simulink library "pmm"  (R2021b)
settings: Solver=VariableStepAuto  StartTime=0.0  StopTime=10.0  RelTol=1e-3
undefined symbols (not defined in the file or in its folder): ENUM_ACMAINRLYSTS_OPEN, ENUM_ACPRECHRGRLYSTS_OPEN, ENUM_B2VRLYSTA_OPEN, ENUM_BMSHVSTS_HVOPEN, ENUM_BRAKEPEDAL_RELEASED, ENUM_CACRLYDEM_CLOSE, ENUM_CACRLYSTS_OPEN, ENUM_CHRGFAULT_ACRLYFAIL, ENUM_CHRGFAULT_BCUHVFAIL, ENUM_CHRGFAULT_BCUNEGFAIL, ENUM_CHRGFAULT_BCUTIMEOUT, ENUM_CHRGFAULT_DCDCENABLE, ENUM_CHRGFAULT_DCDCRLYFAIL, ENUM_CHRGFAULT_HVILFAIL, ENUM_CHRGFAULT_PDUHVFAIL, ENUM_CHRGFAULT_RLYCHKFAIL, ENUM_DCDCEACPCURLYSTA_CLOSED, ENUM_DCDCEACPCURLYSTA_FAILTOCLOSE, ENUM_DCDCEACPCURLYSTA_OPEN, ENUM_DCDCEACPCURLYSTA_WELDED, ENUM_DCDCENABLESTS_READY, ENUM_DCDCRLYSTS_OPEN, ENUM_EHPSRLYDEM_CLOSE, ENUM_EHPSRLYSTS_OPEN, ENUM_FOGRLYENCMD_DISABLE, ENUM_GEARACTUALPOSN_D, ENUM_HVPWROFFREQ_POWEROFF, ENUM_KEYSTATUS_OFF, ENUM_KEYSTATUS_ON, ENUM_KEYSTATUS_START, ENUM_LOWBATTVOLTAGE_NORMAL, ENUM_LOWBATTVOLTAGE_POWERDOWN, ENUM_LOWBATTVOLTAGE_POWERUP, ENUM_MCUHVLOOP_POWEROFF, ENUM_MCUHVLOOPSTS_OPEN, ENUM_MCUMAINRLYSTS_OPEN, ENUM_MCUPRECHRGRLYSTS_OPEN, ENUM_PDFAULT_ACRLYOPEN, ENUM_PDFAULT_BCUDISABLE, ENUM_PDFAULT_DCDCDISABLE, ENUM_PDFAULT_DCDCRLYOPEN, ENUM_PDFAULT_EACDISABLE, ENUM_PDFAULT_EACRLYOPEN, ENUM_PDFAULT_EHPSDISABLE, ENUM_PDFAULT_EHPSRLYOPEN, ENUM_PDFAULT_MCUDISABLE, ENUM_PDFAULT_MCUDISCHRG, ENUM_PDFAULT_MCURLYOPEN, ENUM_PEUSELFCHKSTS_NOFAULT, ENUM_PLUGINSTS_NOPLUGIN, ENUM_PLUGINSTS_PLUGIN, ENUM_PMMMODE_DRIVE, ENUM_PMMMODE_LVBATCHRG, ENUM_PUSTATE_DCDCENABLE, ENUM_PUSTATE_EACPRESCHECK, ENUM_PUSTATE_EHPSENABLE, ENUM_PUSTATE_MCUENABLE, ENUM_PUSTATE_PDUMCURLYCLOSED, ENUM_PUSTATE_POWERUPFAIL, ENUM_TARGETGEAR_REVERSE ... (+126)
libraries: hcu_lib x45, simulink x5, ddm x1, dsc x1
(part 6 of 7)

== stateflow chart pmm/PMM/PowerModeManagement/PMM  ==
  state Sleep
    en:
    VPMM_SysPowerMode_enum = ENUM_PMMMODE_SLEEP;
  state Initialize
    en:
    VPMM_SysPowerMode_enum = ENUM_PMMMODE_INITIALIZE;
    VPMM_IGNRlyClose_flg = FALSE;
    VPMM_IRCRlyClose_flg = FALSE;
    VPMM_PowerUpInhibit_flg = FALSE;
    VPMM_SysInitialTO_flg = FALSE;
    du:
    VPMM_ChrgwakeDebon_cnt += 1;
  state Standby
    en:
    VPMM_SysPowerMode_enum = ENUM_PMMMODE_STANDBY;
    VPMM_PowerUpState_enum = ENUM_PUSTATE_INITIALIZE;
    VPMM_PowerUpFault_enum = ENUM_PUFAULT_NOFAULT;
    VPMM_PowerDownState_enum = ENUM_PDSTATE_MCUDISABLE;
    VPMM_PowerDownFault_enum = ENUM_PDFAULT_NOFAULT;
    VPMM_ChrgState_enum = ENUM_CHRGSTATE_CHECKHVRLYOPEN;
    VPMM_ChrgFault_enum = ENUM_CHRGFAULT_NOFAULT;
    VPMM_PowerUpComplete_flg = FALSE;
    VPMM_PowerDownCompleted_flg = FALSE;
    VPMM_HVSelfChkCompleted_flg = FALSE;
    VPMM_HVSelfChkFail_flg = FALSE;
    VPMM_SysInitialTO_flg = FALSE;
    VPMM_ChrgIntoPwrdown_flg = FALSE;
    VPMM_BattHVDem_enum  = ENUM_BATTHVDEM_POWEROFF;
    VPMM_DCDCRlyDem_enum = ENUM_DCDCRLYDEM_OPEN;
    VPMM_CACRlyDem_enum = ENUM_CACRLYDEM_OPEN;
    VPMM_EHPSRlyDem_enum = ENUM_EHPSRLYDEM_OPEN;
    VPMM_MCUHVLoopDem_enum = ENUM_MCUHVLOOP_POWEROFF;
    VPMM_ACHVLoopDem_enum = ENUM_ACHVLOOP_POWEROFF;
    VPMM_PMMDCDCEnableDem_flg = FALSE;
    VPMM_PMMEACEnableDem_flg = FALSE;
    VPMM_PMMEHPSEnableDem_flg = FALSE;
    VPMM_VCUMCUEn_flg = FALSE;
    VPMM_PowerUpInhibit_flg = FALSE;
    VPMM_DrivelineRelease_enum = ENUM_DRIVELINERELEASE_NOTRELEASE;
    VPMM_ExtTorquePrevent_enum = ENUM_TORQUEPRVENT_NOREQUEST;
    VPMM_HVSysReady_enum = ENUM_HVSYSREADY_NOTREADY;
    VPMM_VCUMCUCtrlMd_enum  = ENUM_MCUCTRLMODE_NONE;
    VPMM_AfterrunCompleted_flg = FALSE;
    (default) -> (junction 1799) : {
        | VPMM_TimeHVSelfChk_s = 0;
        | }
    Standby -> (junction 1799) [order 1]
    (junction 1799) -> (junction 585)
    (junction 585) -> (junction 584) [order 1] : [VINP_ChargeWakeup_flg]
    (junction 584) -> (junction 588) : {
        | VPMM_IRCRlyClose_flg = TRUE;
        | }
    (junction 585) -> (junction 586) [order 2] : {
        | VPMM_IGNRlyClose_flg = TRUE;
        | VPMM_IRCRlyClose_flg = TRUE;
        | }
    (junction 586) -> (junction 587) [order 1] : [VPMM_HVUnitSelfChkCompleted4PU_flg]
    (junction 588) -> (junction 589) [order 1] : [VPMM_HVUnitSelfChkCompleted4Chrg_flg]
    (junction 586) -> (junction 590) [order 2]
    (junction 587) -> (junction 591) : {
        | VPMM_HVSelfChkCompleted4PU_flg =TRUE;
        | }
    (junction 588) -> (junction 1309) [order 2] : {
        | VPMM_TimeHVSelfChk_s += task_time_s;
        | }
    (junction 589) -> (junction 592) : {
        | VPMM_HVSelfChkCompleted4Chrg_flg =TRUE;
        | }
    (junction 591) -> (junction 590)
    (junction 590) -> (junction 596) : {VPMM_TimeHVSelfChk_s += task_time_s;}
    (junction 592) -> (junction 1309)
    (junction 1309) -> (junction 594)
    (junction 594) -> (junction 595) [order 1] : [VPMM_TimeHVSelfChk_s > KPMM_TimeHVSelfChk4Chrg_s]
    (junction 596) -> (junction 597) [order 1] : [VPMM_TimeHVSelfChk_s > KPMM_SysInitialTO_s]
    (junction 594) -> (junction 599) [order 2]
    (junction 595) -> (junction 600) : {
        | VPMM_HVSelfChkFail_flg = TRUE;
        | }
    (junction 596) -> (junction 598) [order 2]
    (junction 597) -> (junction 602) : {
        | VPMM_SysInitialTO_flg = TRUE;
        | }
    (junction 600) -> (junction 599)
    (junction 599) -> (junction 602)
    (junction 602) -> (junction 598)
  state Idle
    en:
    %VPMM_SysPowerMode_enum = ENUM_PMMMODE_IDLE;
    VPMM_PwrOffCompleted_flg = FALSE;
    VPMM_IRCRlyClose_flg =FALSE;
    VPMM_IGNRlyClose_flg = FALSE;
    (default) -> (junction 603) : {
        | VPMM_TimeSysPowerOff_s = 0;
        | }
    Idle -> (junction 603) [order 1]
    (junction 603) -> (junction 604) [order 1] : [((VPMM_TimeSysPowerOff_s > KPMM_Time4Sleep_s) && !VINP_ChargeWakeup_flg) ||...
        |  KPMM_ForceEntrySleep_flg]
    (junction 603) -> (junction 605) [order 2] : {
        | VPMM_TimeSysPowerOff_s += task_time_s;
        | }
    (junction 604) -> (junction 606) : {
        | VPMM_PwrOffCompleted_flg = TRUE;
        | }
    (junction 606) -> (junction 605)
  state Drive
    (default) -> (junction 1819)
    (junction 1819) -> (junction 1821) [order 1] : [VPMM_LVChrgInit2PowerUp_flg || VPMM_LVChrgDCDCDis_flg]
    Drive -> (junction 1819) [order 1]
    (junction 1821) -> (junction 1822) : {
        | VPMM_SysPowerMode_enum = ENUM_PMMMODE_LVBATCHRG;
        | }
    (junction 1819) -> (junction 1823) [order 2] : {
        | VPMM_SysPowerMode_enum = ENUM_PMMMODE_DRIVE;
        | }
    (junction 1822) -> (junction 1823)
    (junction 1823) -> (junction 607)
    (junction 607) -> (junction 608) [order 1] : [(VINP_DCChrgConnectSts_enum ~= ENUM_PLUGINSTS_NOPLUGIN) || (!VINP_MCUIGBTEnFbk_flg) || VPMM_LVChrgInit2PowerUp_flg || VPMM_LVChrgDCDCDis_flg]
    (junction 607) -> (junction 609) [order 2]
    (junction 608) -> (junction 613) : {
        | VPMM_DrivelineRelease_enum = ENUM_DRIVELINERELEASE_NOTRELEASE;
        | }
    (junction 609) -> (junction 610) [order 1] : [VINP_DCChrgConnectSts_enum == ENUM_PLUGINSTS_NOPLUGIN]
    (junction 609) -> (junction 611) [order 2]
    (junction 610) -> (junction 612) : {
        | VPMM_DrivelineRelease_enum = ENUM_DRIVELINERELEASE_RELEASE;
        | }
    (junction 612) -> (junction 611)
    (junction 613) -> (junction 612)
  state Powerdown
    en:
    VPMM_SysPowerMode_enum = ENUM_PMMMODE_POWERDOWN;
    VPMM_HVSysReady_enum = ENUM_HVSYSREADY_NOTREADY;
    VPMM_DrivelineRelease_enum = ENUM_DRIVELINERELEASE_NOTRELEASE;
    VPMM_PowerDownCompleted_flg = FALSE;
    state Initialize
      en:
      VPMM_PowerDownFault_enum = ENUM_PDFAULT_NOFAULT;
      VPMM_PowerDownCompleted_flg = FALSE;
      VPMM_HVSysReady_enum = ENUM_HVSYSREADY_NOTREADY;
      VPMM_DrivelineRelease_enum = ENUM_DRIVELINERELEASE_NOTRELEASE;
      VPMM_MCUDisableCompleted_flg = FALSE;
      VPMM_PDUDisableCompleted_flg = FALSE;
      VPMM_BattPDCompleted_flg = FALSE;
      VPMM_BattPackPDFail_flg = FALSE;
      VPMM_MCUDisChrgCompleted_flg=FALSE;
      VPMM_MCUDisChrgFail_flg = FALSE;
      VPMM_MCUEnDischrgCompleted_flg = FALSE;
      VPMM_MCUEnDischrgFail_flg = FALSE;
      VPMM_MCUPassDischrgFinish_flg = FALSE;
      VPMM_PDURLYOpenFinish_flg = FALSE;
      VPMM_PDURLYOpenFinishFM_flg = FALSE;
      VPMM_ForcedPowerDown4IRC_flg = FALSE;
    state MCUDisable
      en:
      VPMM_PowerDownState_enum = ENUM_PDSTATE_MCUDISABLE;
      VPMM_MCUDisableCompleted_flg = FALSE;
      VPMM_TimeMCUDisable_s = 0;
      (default) -> (junction 773) : {
          | VPMM_VCUMCUEn_flg = FALSE;
          | }
      MCUDisable -> (junction 773) [order 1]
      (junction 773) -> (junction 774) [order 1] : [VINP_MCUIGBTEnFbk_flg == FALSE]
      (junction 773) -> (junction 775) [order 2] : {VPMM_TimeMCUDisable_s += task_time_s}
      (junction 774) -> (junction 779) : {
          | VPMM_MCUDisableCompleted_flg = TRUE;
          | }
      (junction 775) -> (junction 776) [order 1] : [VPMM_TimeMCUDisable_s > KPMM_MCUDisableFailtime_s]
      (junction 776) -> (junction 778) : {
          | VPMM_PowerDownFault_enum = ENUM_PDFAULT_MCUDISABLE;
          | VPMM_MCUDisableCompleted_flg = TRUE;
          | }
      (junction 775) -> (junction 777) [order 2]
      (junction 778) -> (junction 777)
      (junction 779) -> (junction 778)
    state PEUDisable
      en:
      VPMM_PowerDownState_enum = ENUM_PDSTATE_PDUDISABLE;
      VPMM_PDUDisableCompleted_flg = FALSE;
      VPMM_TimePDUDisable_s = 0;
      VPMM_TimePDUDisableWait_s = 0;
      VPMM_DCDCDisableFail_flg = FALSE;
      VPMM_EHPSDisableFail_flg = FALSE;
      VPMM_EACDisableFail_flg = FALSE;
      (default) -> (junction 723) : {
          | VPMM_PMMDCDCEnableDem_flg = FALSE;
          | VPMM_PMMEACEnableDem_flg = FALSE;
          | VPMM_PMMEHPSEnableDem_flg = FALSE;
          | }
      PEUDisable -> (junction 723) [order 1]
      (junction 723) -> (junction 724) [order 1] : [
          |  ((VINP_DCDCEnableStatus_enum == ENUM_DCDCENABLESTS_READY) || (VINP_DCDCEnableStatus_enum == ENUM_DCDCENABLESTS_INITIAL)) &&...
          |  ((VINP_EHPSEnableStatus_enum == ENUM_EHPSENABLESTS_READY)  || (VINP_EHPSEnableStatus_enum == ENUM_EHPSENABLESTS_INITIAL)) &&...
          |  ((VINP_EACEnSta_enum == ENUM_CACENABLESTS_READY) || (VINP_EACEnSta_enum == ENUM_CACENABLESTS_INITIAL))
          | ]
      (junction 723) -> (junction 725) [order 2] : {VPMM_TimePDUDisable_s += task_time_s}
      (junction 724) -> (junction 742) : {
          | VPMM_PDUDisableCompleted_flg = TRUE;
          | }
      (junction 725) -> (junction 726) [order 1] : [VPMM_TimePDUDisable_s > KPMM_PDUDisableFailtime_s]
      (junction 725) -> (junction 739) [order 2]
      (junction 726) -> (junction 727) : {VPMM_TimePDUDisableWait_s += task_time_s}
      (junction 727) -> (junction 1305) [order 1] : [
          |  ((VINP_DCDCEnableStatus_enum == ENUM_DCDCENABLESTS_RUN) ||(VINP_DCDCEnableStatus_enum == ENUM_DCDCENABLESTS_FAULT)) &&...
          |  (VPMM_DCDCDisableFail_flg == FALSE)
          | ]
      (junction 727) -> (junction 729) [order 2]
      (junction 1305) -> (junction 735) : {
          | VPMM_DCDCDisableFail_flg = TRUE;
          | VPMM_PowerDownFault_enum = ENUM_PDFAULT_DCDCDISABLE;
          | }
      (junction 729) -> (junction 1303) [order 1] : [
          | ((VINP_EHPSEnableStatus_enum == ENUM_EHPSENABLESTS_RUN) || (VINP_EHPSEnableStatus_enum == ENUM_EHPSENABLESTS_FAULT)) && ...
          | (VPMM_EHPSDisableFail_flg == FALSE)
          | ]
      (junction 729) -> (junction 731) [order 2]
      (junction 1303) -> (junction 734) : {
          | VPMM_EHPSDisableFail_flg = TRUE;
          | VPMM_PowerDownFault_enum = ENUM_PDFAULT_EHPSDISABLE;
          | }
      (junction 731) -> (junction 732) [order 1] : [
          | ((VINP_EACEnSta_enum == ENUM_CACENABLESTS_RUN) || (VINP_EACEnSta_enum == ENUM_CACENABLESTS_FAULT)) && ...
          | (VPMM_EACDisableFail_flg == FALSE)
          | ]
      (junction 732) -> (junction 733) : {
          | VPMM_EACDisableFail_flg = TRUE;
          | VPMM_PowerDownFault_enum = ENUM_PDFAULT_EACDISABLE;
          | }
      (junction 731) -> (junction 736) [order 2]
      (junction 734) -> (junction 733)
      (junction 735) -> (junction 734)
      (junction 733) -> (junction 736)
      (junction 736) -> (junction 737)
      (junction 737) -> (junction 738) [order 1] : [VPMM_TimePDUDisableWait_s > KPMM_PDUDisableWaitime_s]
      (junction 737) -> (junction 740) [order 2]
      (junction 738) -> (junction 741) : {
          | VPMM_PDUDisableCompleted_flg = TRUE;
          | }
      (junction 740) -> (junction 739)
      (junction 741) -> (junction 740)
      (junction 742) -> (junction 741)
    state HVRelayOpen
      en:
      VPMM_PowerDownState_enum = ENUM_PDSTATE_PDURLYOPEN;
      VPMM_PDURLYOpenFinish_flg = FALSE;
      VPMM_TimeHVRlyOpen_s = 0;
      VPMM_TimeHVRlyOpenWait_s = 0;
      VPMM_PDURLYOpenFail_flg = FALSE;
      VPMM_EHPSRlyOpenFail_flg = FALSE;
      VPMM_ACRlyOpenFail_flg = FALSE;
      VPMM_EACRlyOpenFail_flg = FALSE;
      VPMM_DCDCRlyOpenFail_flg = FALSE;
      VPMM_MainRlyOpenFail_flg = FALSE;
      (default) -> (junction 838) : {
          | VPMM_MCUHVLoopDem_enum = ENUM_MCUHVLOOP_POWEROFF;
          | VPMM_DCDCRlyDem_enum = ENUM_DCDCRLYDEM_OPEN;
          | VPMM_CACRlyDem_enum = ENUM_CACRLYDEM_OPEN;
          | VPMM_EHPSRlyDem_enum = ENUM_EHPSRLYDEM_OPEN;
          | VPMM_ACHVLoopDem_enum = ENUM_ACHVLOOP_POWEROFF;
          | }
      (junction 838) -> (junction 839) [order 1] : [
          | (VINP_MCUHVLoopSts_enum == ENUM_MCUHVLOOPSTS_OPEN &&...
          | VPMM_PDUDCDCRlySta_enum == ENUM_DCDCRLYSTS_OPEN &&...
          | VPMM_PDUEACRlySta_enum == ENUM_CACRLYSTS_OPEN &&...
          | VPMM_PDUEHPSRlySta_enum == ENUM_EHPSRLYSTS_OPEN &&...
          | VINP_PDUACRlySta_enum== ENUM_PDUACRLYSTA_OPEN &&...
          | VINP_PDUACRlySta_enum == ENUM_ACMAINRLYSTS_OPEN &&...
          | VINP_PDUMCUPosRlySta_enum == ENUM_MCUMAINRLYSTS_OPEN) && ...
          | ~VPMM_PDURLYOpenFail_flg
          | ]
      HVRelayOpen -> (junction 838) [order 1]
      (junction 838) -> (junction 840) [order 2] : {
          | VPMM_TimeHVRlyOpen_s += task_time_s;
          | }
      (junction 839) -> (junction 852)
      (junction 840) -> (junction 841) [order 1] : [VPMM_TimeHVRlyOpen_s > KPMM_HVRlyOpenFailtime_s]
      (junction 840) -> (junction 866) [order 2]
      (junction 841) -> (junction 842) : {
          | VPMM_TimeHVRlyOpenWait_s += task_time_s;
          | VPMM_PDURLYOpenFail_flg = TRUE;
          | }
      (junction 842) -> (junction 843) [order 1] : [(VPMM_PDUEHPSRlySta_enum ~= ENUM_EHPSRLYSTS_OPEN) && ...
          |  (VPMM_EHPSRlyOpenFail_flg == FALSE)]
      (junction 842) -> (junction 844) [order 2]
      (junction 843) -> (junction 859) : {
          | VPMM_EHPSRlyOpenFail_flg = TRUE;
          | VPMM_PowerDownFault_enum = ENUM_PDFAULT_EHPSRLYOPEN;
          | }
      (junction 844) -> (junction 845) [order 1] : [((VINP_PDUACRlySta_enum~= ENUM_PDUACRLYSTA_OPEN) || ...
          |   (VINP_PDUACRlySta_enum ~= ENUM_ACMAINRLYSTS_OPEN)) && ...
          |   (VPMM_ACRlyOpenFail_flg == FALSE)]
      (junction 844) -> (junction 846) [order 2]
      (junction 845) -> (junction 858) : {
          | VPMM_ACRlyOpenFail_flg = TRUE;
          | VPMM_PowerDownFault_enum = ENUM_PDFAULT_ACRLYOPEN;
          | }
      (junction 846) -> (junction 847) [order 1] : [(VPMM_PDUEACRlySta_enum ~= ENUM_CACRLYSTS_OPEN) &&...
          |  (VPMM_EACRlyOpenFail_flg == FALSE)]
      (junction 846) -> (junction 848) [order 2]
      (junction 847) -> (junction 857) : {
          | VPMM_EACRlyOpenFail_flg = TRUE;
          | VPMM_PowerDownFault_enum = ENUM_PDFAULT_EACRLYOPEN;
          | }
      (junction 848) -> (junction 849) [order 1] : [(VPMM_PDUDCDCRlySta_enum ~= ENUM_DCDCRLYSTS_OPEN) && ...
          |  (VPMM_DCDCRlyOpenFail_flg == FALSE)]
      (junction 848) -> (junction 850) [order 2]
      (junction 849) -> (junction 856) : {
          | VPMM_DCDCRlyOpenFail_flg = TRUE;
          | VPMM_PowerDownFault_enum = ENUM_PDFAULT_DCDCRLYOPEN;
          | }
      (junction 850) -> (junction 851) [order 1] : [((VINP_MCUHVLoopSts_enum ~= ENUM_MCUHVLOOPSTS_OPEN) || ...
          |  (VINP_PDUMCUPosRlySta_enum ~= ENUM_MCUMAINRLYSTS_OPEN)) && ...
          |  (VPMM_MainRlyOpenFail_flg == FALSE)]
      (junction 850) -> (junction 854) [order 2]
      (junction 851) -> (junction 855) : {
          | VPMM_MainRlyOpenFail_flg = TRUE;
          | VPMM_PowerDownFault_enum = ENUM_PDFAULT_MCURLYOPEN;
          | }
      (junction 852) -> (junction 853) [order 1] : [VPMM_BattPackPDFail_flg]
      (junction 852) -> (junction 868) [order 2] : {
          | VPMM_PDURLYOpenFinish_flg = TRUE;
          | }
      (junction 853) -> (junction 869) : {
          | VPMM_PDURLYOpenFinishFM_flg = TRUE;
          | }
      (junction 855) -> (junction 854)
      (junction 856) -> (junction 855)
      (junction 857) -> (junction 856)
      (junction 858) -> (junction 857)
      (junction 859) -> (junction 858)
      (junction 854) -> (junction 860)
      (junction 860) -> (junction 861) [order 1] : [VPMM_TimeHVRlyOpenWait_s > KPMM_HVRlyOpenFailWT_s]
      (junction 860) -> (junction 867) [order 2]
      (junction 861) -> (junction 862)
      (junction 862) -> (junction 863) [order 1] : [VPMM_BattPackPDFail_flg]
      (junction 862) -> (junction 864) [order 2] : {
          | VPMM_PDURLYOpenFinish_flg = TRUE;
          | }
      (junction 863) -> (junction 865) : {
          | VPMM_PDURLYOpenFinishFM_flg = TRUE;
          | }
      (junction 865) -> (junction 864)
      (junction 868) -> (junction 865)
      (junction 864) -> (junction 867)
      (junction 867) -> (junction 866)
      (junction 869) -> (junction 868)
    state BCUPowerDown
      en:
      VPMM_PowerDownState_enum = ENUM_PDSTATE_BCUPWRDOWN;
      VPMM_BattPDCompleted_flg = FALSE;
      VPMM_BattPackPDFail_flg = FALSE;
      VPMM_TimeBattPD_s = 0;
      (default) -> (junction 750) : {
          | VPMM_BattHVDem_enum  = ENUM_BATTHVDEM_POWEROFF;
          | }
      BCUPowerDown -> (junction 750) [order 1]
      (junction 750) -> (junction 751) [order 1] : [VINP_BMSHVSts_enum == ENUM_BMSHVSTS_HVOPEN]
      (junction 750) -> (junction 752) [order 2] : {
          | VPMM_TimeBattPD_s += task_time_s;
          | }
      (junction 751) -> (junction 756) : {
          | VPMM_BattPDCompleted_flg = TRUE;
          | }
      (junction 752) -> (junction 753) [order 1] : [(VPMM_TimeBattPD_s > KPMM_BattDownFailtime_s)]
      (junction 753) -> (junction 755) : {
          | VPMM_PowerDownFault_enum = ENUM_PDFAULT_BCUDISABLE;
          | VPMM_BattPackPDFail_flg = TRUE;
          | }
      (junction 752) -> (junction 754) [order 2]
      (junction 755) -> (junction 754)
      (junction 756) -> (junction 755)
    state MCUDischarge
      en:
      VPMM_PowerDownState_enum = ENUM_PDSTATE_MCUDISCHRG;
      VPMM_MCUDisChrgCompleted_flg=FALSE;
      VPMM_MCUDisChrgFail_flg = FALSE;
      VPMM_TimeMCUDisChrg_s = 0;
      VPMM_AtvDisChgEnFbkLatch_flg = FALSE;
      (default) -> (junction 1839) : {
          | VPMM_VCUMCUCtrlMd_enum = ENUM_MCUCTRLMODE_ACTDISCHRG;
          | }
      (junction 1839) -> (junction 1841)
      MCUDischarge -> (junction 1841) [order 1]
      (junction 1841) -> (junction 1843) [order 1] : [VPMM_AtvDisChgEnFbk_flg]
      (junction 1841) -> (junction 1847) [order 2]
      (junction 1843) -> (junction 1845) : {
          | VPMM_AtvDisChgEnFbkLatch_flg = TRUE;
          | }
      (junction 1845) -> (junction 1847)
      (junction 1847) -> (junction 757)
      (junction 757) -> (junction 758) [order 1] : [((VINP_MCUInVol_V < KPMM_TargetDchrgVolt_V) && VPMM_AtvDisChgEnFbkLatch_flg )|| VPMM_ChrgIntoPwrdown_flg]
      (junction 757) -> (junction 759) [order 2] : {
          | VPMM_TimeMCUDisChrg_s += task_time_s;
          | }
      (junction 758) -> (junction 763) : {
          | VPMM_VCUMCUCtrlMd_enum = ENUM_MCUCTRLMODE_NONE;
          | VPMM_MCUDisChrgCompleted_flg = TRUE;
          | }
      (junction 759) -> (junction 760) [order 1] : [VPMM_TimeMCUDisChrg_s > KPMM_MCUDisChrgFailtime_s]
      (junction 759) -> (junction 761) [order 2]
      (junction 760) -> (junction 762) : {
          | VPMM_PowerDownFault_enum = ENUM_PDFAULT_MCUDISCHRG;
          | VPMM_VCUMCUCtrlMd_enum = ENUM_MCUCTRLMODE_NONE;
          | VPMM_MCUDisChrgFail_flg = TRUE;
          | }
      (junction 762) -> (junction 761)
      (junction 763) -> (junction 762)
    state MCUDischarge_FailMode
      en:
      VPMM_PowerDownState_enum = ENUM_PDSTATE_MCUDISCHRGFS;
      VPMM_TimeMCUEnDisChrg_s  = 0;
      VPMM_TimeMCUDisable_s = 0;
      VPMM_MCUEnDischrgCompleted_flg = FALSE;
      VPMM_MCUEnDischrgFailCom_flg = FALSE;
      VPMM_MCUEnDischrgFinish_flg = FALSE;
      VPMM_MCUEnFailDis_flg = FALSE;
      (default) -> (junction 819) : {
          | VPMM_VCUMCUEn_flg = TRUE;
          | }
      MCUDischarge_FailMode -> (junction 819) [order 3]
      (junction 819) -> (junction 820) [order 1] : [VINP_MCUInVol_V < KPMM_TargetEnDischrgVolt_V]
      MCUDischarge_FailMode -> (junction 820) [order 1] : [VPMM_MCUEnDischrgFinish_flg == TRUE]
      (junction 819) -> (junction 821) [order 2] : {
          | VPMM_TimeMCUEnDisChrg_s += task_time_s;
          | }
      (junction 820) -> (junction 825) : {
          | VPMM_VCUMCUEn_flg = FALSE;
          | VPMM_MCUEnDischrgFinish_flg = TRUE;
          | }
      MCUDischarge_FailMode -> (junction 821) [order 2] : [VPMM_MCUEnFailDis_flg == TRUE]
      (junction 821) -> (junction 822) [order 1] : [VPMM_TimeMCUEnDisChrg_s > KPMM_MCUEnDischrgFailtime_s]
      (junction 821) -> (junction 831) [order 2]
      (junction 822) -> (junction 823) : {
          | VPMM_VCUMCUEn_flg = FALSE;
          | VPMM_MCUEnFailDis_flg = TRUE;
          | }
      (junction 823) -> (junction 824) [order 1] : [VINP_MCUIGBTEnFbk_flg == FALSE]
      (junction 825) -> (junction 826) [order 1] : [VINP_MCUIGBTEnFbk_flg == FALSE]
      (junction 823) -> (junction 829) [order 2] : {
          | VPMM_TimeMCUDisable_s += task_time_s;
          | }
      (junction 824) -> (junction 834) : {
          | VPMM_MCUEnDischrgFail_flg = TRUE;
          | }
      (junction 825) -> (junction 827) [order 2] : {
          | VPMM_TimeMCUDisable_s += task_time_s;
          | }
      (junction 826) -> (junction 837) : {
          | VPMM_MCUEnDischrgCompleted_flg = TRUE;
          | }
      (junction 827) -> (junction 828) [order 1] : [VPMM_TimeMCUDisable_s > KPMM_MCUDisableFailtime_s]
      (junction 827) -> (junction 835) [order 2]
      (junction 828) -> (junction 836) : {
          | VPMM_PowerDownFault_enum = ENUM_PDFAULT_MCUDISABLE;
          | VPMM_MCUEnDischrgCompleted_flg = TRUE;
          | }
      (junction 829) -> (junction 830) [order 1] : [VPMM_TimeMCUDisable_s > KPMM_MCUDisableFailtime_s]
      (junction 829) -> (junction 832) [order 2]
      (junction 830) -> (junction 833) : {
          | VPMM_PowerDownFault_enum = ENUM_PDFAULT_MCUDISABLE;
          | VPMM_MCUEnDischrgFailCom_flg = TRUE;
          | }
      (junction 832) -> (junction 831)
      (junction 833) -> (junction 832)
      (junction 834) -> (junction 833)
      (junction 835) -> (junction 834)
      (junction 836) -> (junction 835)
      (junction 837) -> (junction 836)
    state BCU_FailMode
      en:
      VPMM_PowerDownState_enum = ENUM_PDSTATE_BCUNEGRLUFS;
      VPMM_MainRlyOpenCompleted_flg = FALSE;
      VPMM_MCUDisChrgFail_flg = FALSE;
      VPMM_TimeMCUDisChrg_s = 0;
      (default) -> (junction 796) : {
          | VPMM_VCUMCUCtrlMd_enum = ENUM_MCUCTRLMODE_ACTDISCHRG;
          | }
      BCU_FailMode -> (junction 796) [order 1]
      (junction 796) -> (junction 797) [order 1] : [VINP_MCUInVol_V < KPMM_TargetDchrgVolt_V]
      (junction 797) -> (junction 802) : {
          | VPMM_VCUMCUCtrlMd_enum = ENUM_MCUCTRLMODE_NONE;
          | VPMM_MCUDisChrgCompleted_flg = TRUE;
          | }
      (junction 796) -> (junction 798) [order 2] : {
          | VPMM_TimeMCUDisChrg_s += task_time_s;
          | }
      (junction 798) -> (junction 799) [order 1] : [VPMM_TimeMCUDisChrg_s > KPMM_MCUDisChrgFSFailtime_s]
      (junction 798) -> (junction 800) [order 2]
      (junction 799) -> (junction 801) : {
          | VPMM_PowerDownFault_enum = ENUM_PDFAULT_MCUDISCHRG;
          | VPMM_VCUMCUCtrlMd_enum = ENUM_MCUCTRLMODE_NONE;
          | VPMM_MCUDisChrgFail_flg = TRUE;
          | }
      (junction 801) -> (junction 800)
      (junction 802) -> (junction 801)
    state MCUPassiveDischrg
      en:
      VPMM_PowerDownState_enum = ENUM_PDSTATE_MCUPASSDISCHRG;
      VPMM_TimeMCUPassDisChrg_s = 0;
      VPMM_MCUPassDischrgFinish_flg = FALSE;
      (default) -> (junction 870)
      MCUPassiveDischrg -> (junction 870) [order 1]
      (junction 870) -> (junction 871) [order 1] : [VINP_MCUInVol_V < KPMM_TargetPassDischrgVolt_V]
      (junction 870) -> (junction 872) [order 2] : {VPMM_TimeMCUPassDisChrg_s += task_time_s}
      (junction 871) -> (junction 876) : {
          | VPMM_MCUPassDischrgFinish_flg = TRUE;
          | }
      (junction 872) -> (junction 873) [order 1] : [VPMM_TimeMCUPassDisChrg_s > KPMM_MCUPassDisChrg_s]
      (junction 872) -> (junction 874) [order 2]
      (junction 873) -> (junction 875) : {
          | VPMM_MCUPassDischrgFinish_flg = TRUE;
          | }
      (junction 875) -> (junction 874)
      (junction 876) -> (junction 875)
    state PowerDownCompleted
      en:
      VPMM_PowerDownState_enum = ENUM_PDSTATE_PDCOMPLETED;
      VPMM_PowerDownCompleted_flg = TRUE;
    state PowerdownFailSafeFinished
      en:
      VPMM_PowerDownState_enum = ENUM_PDSTATE_FSCOMPLETED;
      VPMM_PowerDownCompleted_flg = TRUE;
    (default) -> Powerdown.Initialize
    Powerdown.Initialize -> MCUDisable
    MCUDisable -> PEUDisable [order 1] : [VPMM_MCUDisableCompleted_flg]
    PEUDisable -> BCUPowerDown [order 1] : [VPMM_PDUDisableCompleted_flg]
    BCUPowerDown -> HVRelayOpen [order 1] : [VPMM_BattPackPDFail_flg || VDMM_DTCBMSRlyNoFB_flg]
    BCUPowerDown -> MCUDischarge [order 2] : [VPMM_BattPDCompleted_flg]
    MCUDischarge -> HVRelayOpen [order 2] : [VPMM_MCUDisChrgCompleted_flg ||...
        | VPMM_ChrgState_enum != ENUM_CHRGSTATE_CHECKHVRLYOPEN ||...
        | VPMM_ChrgIntoPwrdown_flg]
    MCUDischarge -> MCUDischarge_FailMode [order 1] : [VPMM_MCUDisChrgFail_flg ||...
        | VDMM_DTCMCUCtrlMdNoFB_flg]
    MCUDischarge_FailMode -> HVRelayOpen [order 2] : [VPMM_MCUEnDischrgCompleted_flg]
    MCUDischarge_FailMode -> MCUPassiveDischrg [order 1] : [VPMM_MCUEnDischrgFailCom_flg ||...
        | VPMM_MCUEnDischrgFail_flg]
    HVRelayOpen -> BCU_FailMode [order 1] : [VPMM_PDURLYOpenFinishFM_flg]
    BCU_FailMode -> MCUPassiveDischrg [order 1] : [VPMM_MCUDisChrgFail_flg]
    MCUPassiveDischrg -> PowerdownFailSafeFinished [order 1] : [VPMM_MCUPassDischrgFinish_flg]
    BCU_FailMode -> PowerdownFailSafeFinished [order 2] : [VPMM_MCUDisChrgCompleted_flg]
    HVRelayOpen -> (junction 1486) [order 2]
    HVRelayOpen -> PowerDownCompleted [order 3] : [VPMM_PDURLYOpenFinish_flg]
    (junction 1486) -> PowerdownFailSafeFinished : [VPMM_PDURLYOpenFinish_flg &&...
        | VPMM_MCUEnDischrgCompleted_flg]
  state Powerup
    en:
    VPMM_SysPowerMode_enum = ENUM_PMMMODE_POWERUP;
    VPMM_PowerUpComplete_flg = FALSE;
    VPMM_HVPwrFail_flg  = FALSE;
    state Initialize
      en:
      VPMM_PowerUpState_enum = ENUM_PUSTATE_DRIVESAFE;
      VPMM_PowerUpFault_enum = ENUM_PUFAULT_NOFAULT;
      VPMM_HVRlyCheckCompleted_flg = FALSE;
      VPMM_BattPUCompleted_flg = FALSE;
      VPMM_EHPSEACReady_flg =FALSE;
      VPMM_MCUPrechrgCompleted_flg = FALSE;
      VPMM_HVSysReady_enum = ENUM_HVSYSREADY_NOTREADY;
      VPMM_DrivelineRelease_enum = ENUM_DRIVELINERELEASE_NOTRELEASE;
      VPMM_PowerUpFail_flg = FALSE;
      VPMM_MCUEnableCompleted_flg = FALSE;
      VPMM_PDULoadPUFault_enum = ENUM_PUFAULT_NOFAULT;
    state AlcLockcheck
      en:
      VPMM_PowerUpState_enum = ENUM_PUSTATE_DRIVESAFE;
      (default) -> (junction 1328) : {
          | VPMM_TimeAlcLockCheck_s = 0;
          | }
      AlcLockcheck -> (junction 1328) [order 1]
      (junction 1328) -> (junction 1329)
      (junction 1329) -> (junction 1330) [order 1] : [VPSA_AlcLockPass_flg]
      (junction 1329) -> (junction 1331) [order 2] : {
          | VPMM_TimeAlcLockCheck_s += task_time_s;
          | }
      (junction 1330) -> (junction 1332) : {
          | VPMM_AlcLockCheckCompleted_flg = TRUE;
          | }
      (junction 1332) -> (junction 1331)
    state HVRlycheck
      en:
      VPMM_PowerUpState_enum = ENUM_PUSTATE_HVRLYCHECK;
      (default) -> (junction 768) : {
          | VPMM_TimeHVRlyCheck_s = 0;
          | VPMM_HVRlyCheckCompleted_flg = FALSE;
          | VPMM_BattHVDem_enum = ENUM_BATTHVDEM_POWEROFF;
          | VPMM_DCDCRlyDem_enum = ENUM_DCDCRLYDEM_OPEN;
          | VPMM_EHPSRlyDem_enum = ENUM_EHPSRLYDEM_OPEN;
          | VPMM_CACRlyDem_enum = ENUM_CACRLYDEM_OPEN;
          | VPMM_MCUHVLoopDem_enum = ENUM_MCUHVLOOP_POWEROFF;
          | VPMM_ACHVLoopDem_enum = ENUM_ACHVLOOP_POWEROFF;
          | }
      HVRlycheck -> (junction 768) [order 1]
      (junction 768) -> (junction 769)
      (junction 769) -> (junction 770) [order 1] : [VPMM_RlyOpenCheck_flg]
      (junction 769) -> (junction 771) [order 2] : {
          | VPMM_TimeHVRlyCheck_s += task_time_s;
          | }
      (junction 770) -> (junction 772) : {
          | VPMM_HVRlyCheckCompleted_flg = TRUE;
          | }
      (junction 772) -> (junction 771)
    state HVPwrUpProcess
      en:
      VPMM_BattPUCompleted_flg = FALSE;
      VPMM_DCDCRlyUpCompleted_flg = FALSE;
      VPMM_PDURelayPUReady_flg = FALSE;
      VPMM_MCUPrechrgCompleted_flg = FALSE;
      VPMM_DCDCEnableCompleted_flg = FALSE;
      VPMM_MCUEnableCompleted_flg  = FALSE;
      VPMM_PowerUpComplete_flg = FALSE;
      VPMM_HVPwrFail_flg  = FALSE;
      VPMM_DCDCEnableProc_flg = FALSE;
      VPMM_MCUPrechrgProc_flg = FALSE;
      VPMM_MCUEnableProc_flg = FALSE;
      VPMM_EHPSEnableProc_flg = FALSE;
      VPMM_CACPresReadyProc_flg = FALSE;
      VPMM_PMMEHPSEnableDem_flg = FALSE;
      VPMM_EHPSEnableCompleted_flg = FALSE;
      VPMM_EHPSIniFinish_flg = FALSE;
      VPMM_PMMEACEnableDem_flg = FALSE;
      VPMM_EACEnableCompleted_flg = FALSE;
      VPMM_AirPressReady_flg = FALSE;
      state BattPackPowerup
        en:
        VPMM_PowerUpState_enum = ENUM_PUSTATE_BCUPOSRLYCLOSED;
        VPMM_BattPUCompleted_flg = FALSE;
        (default) -> (junction 685) : {
            | VPMM_TimeBattPU_s = 0;
            | }
        BattPackPowerup -> (junction 685) [order 1]
        (junction 685) -> (junction 686) : {
            | VPMM_BattHVDem_enum = ENUM_BATTHVDEM_POWERON;
            | }
        (junction 686) -> (junction 687) [order 1] : [VINP_BMSHVSts_enum == ENUM_BMSHVSTS_HVCLOSED]
        (junction 686) -> (junction 688) [order 2] : {
            | VPMM_TimeBattPU_s += task_time_s;
            | }
        (junction 687) -> (junction 689) : {
            | VPMM_BattPUCompleted_flg = TRUE;
            | }
        (junction 689) -> (junction 688)
      state DCDCRlyClosed
        en:
        VPMM_PowerUpState_enum = ENUM_PUSTATE_DCDCRLYCLOSED;
        VPMM_DCDCRlyUpCompleted_flg = FALSE;
        (default) -> (junction 878) : {
            | VPMM_TimeDCDCRlyDemDelay_s = 0;
            | VPMM_TimeDCDCRlyPU_s = 0;
            | }
        Powerup.HVPwrUpProcess.DCDCRlyClosed -> (junction 878) [order 1]
        (junction 878) -> (junction 879) [order 1] : [VPMM_TimeDCDCRlyDemDelay_s > KPMM_DCDCRlyDemDelayTime_s]
        (junction 878) -> (junction 882) [order 2] : {
            | VPMM_TimeDCDCRlyDemDelay_s += task_time_s;
            | }
        (junction 879) -> (junction 880) : {
            | VPMM_DCDCRlyDem_enum = ENUM_DCDCRLYDEM_CLOSE;
            | }
        (junction 880) -> (junction 881) [order 1] : [VPMM_PDUDCDCRlySta_enum == ENUM_DCDCRLYSTS_CLOSED]
        (junction 880) -> (junction 883) [order 2] : {
            | VPMM_TimeDCDCRlyPU_s += task_time_s;
            | }
        (junction 881) -> (junction 884) : {
            | VPMM_DCDCRlyUpCompleted_flg = TRUE;
            | }
        (junction 882) -> (junction 883)
        (junction 884) -> (junction 883)
      state PDULoadRlyClosed
        en:
        VPMM_PowerUpState_enum = ENUM_PUSTATE_PDURLYCLOSED;
        VPMM_CACRlyUpCompleted_flg = FALSE;
        VPMM_EHPSRlyUpCompleted_flg = FALSE;
        VPMM_ACMainRlyUpCompleted_flg = FALSE;
        VPMM_PDURelayPUReady_flg = FALSE;
        (default) -> (junction 885) : {
            | VPMM_TimePDULoadRlyPU_s = 0;
            | }
        PDULoadRlyClosed -> (junction 885) [order 1]
        (junction 885) -> (junction 886) : {
            | VPMM_CACRlyDem_enum = ENUM_CACRLYDEM_CLOSE;
            | VPMM_EHPSRlyDem_enum = ENUM_EHPSRLYDEM_CLOSE;
            | VPMM_ACHVLoopDem_enum = ENUM_ACHVLOOP_POWERON;
            | }
        (junction 886) -> (junction 887) [order 1] : [VPMM_PDUEACRlySta_enum == ENUM_CACRLYSTS_CLOSED]
        (junction 886) -> (junction 888) [order 2]
        (junction 887) -> (junction 889) : {
            | VPMM_CACRlyUpCompleted_flg = TRUE;
            | }
        (junction 889) -> (junction 888)
        (junction 888) -> (junction 890)
        (junction 890) -> (junction 891) [order 1] : [VPMM_PDUEHPSRlySta_enum == ENUM_EHPSRLYSTS_CLOSED]
        (junction 890) -> (junction 892) [order 2]
        (junction 891) -> (junction 893) : {
            | VPMM_EHPSRlyUpCompleted_flg = TRUE;
            | }
        (junction 893) -> (junction 892)
        (junction 892) -> (junction 894)
        (junction 894) -> (junction 895) [order 1] : [VINP_PDUACRlySta_enum ==ENUM_PDUACRLYSTA_CLOSE]
        (junction 894) -> (junction 896) [order 2]
        (junction 895) -> (junction 897) : {
            | VPMM_ACMainRlyUpCompleted_flg = TRUE;
            | }
        (junction 897) -> (junction 896)
        (junction 896) -> (junction 898)
        (junction 898) -> (junction 899) [order 1] : [VPMM_ACMainRlyUpCompleted_flg && VPMM_EHPSRlyUpCompleted_flg && VPMM_CACRlyUpCompleted_flg]
        (junction 898) -> (junction 900) [order 2] : {
            | VPMM_TimePDULoadRlyPU_s += task_time_s;
            | }
        (junction 899) -> (junction 901) : {
            | VPMM_PDURelayPUReady_flg = TRUE;
            | }
        (junction 901) -> (junction 900)
        (junction 900) -> (junction 902)
      state HVPwrEnable
        state MCU [parallel]
          settings: executionOrder=1
          state MCUPrechrg
            en:
            VPMM_MCUPrechrgCompleted_flg = FALSE;
            VPMM_PowerUpState_enum = ENUM_PUSTATE_PDUMCURLYCLOSED;
            VPMM_MCUPrechrgProc_flg = TRUE;
            exit:
            VPMM_MCUPrechrgProc_flg = FALSE;
            (default) -> (junction 908) : {
                | VPMM_TimeMCUPrechrgRlyPU_s = 0;
                | }
            MCUPrechrg -> (junction 908) [order 1]
            (junction 908) -> (junction 909) [order 1] : [VINP_MCUFailGrade_enum == ZERO_INT]
            (junction 909) -> (junction 910) : {
                | VPMM_MCUHVLoopDem_enum = ENUM_MCUHVLOOP_POWERON;
                | }
            (junction 908) -> (junction 912) [order 2] : {
                | VPMM_TimeMCUPrechrgRlyPU_s += task_time_s;
                | }
            (junction 910) -> (junction 911) [order 1] : [VINP_MCUHVLoopSts_enum == ENUM_MCUHVLOOPSTS_PRECHARGEFIN]
            (junction 911) -> (junction 914) : {
                | VPMM_MCUPrechrgCompleted_flg = TRUE;
                | }
            (junction 910) -> (junction 913) [order 2] : {
                | VPMM_TimeMCUPrechrgRlyPU_s += task_time_s;
                | }
            (junction 913) -> (junction 912)
            (junction 914) -> (junction 913)
          state MCUEnable
            en:
            VPMM_MCUEnableCompleted_flg  = FALSE;
            VPMM_PowerUpState_enum = ENUM_PUSTATE_MCUENABLE;
            VPMM_MCUEnableProc_flg = TRUE;
            exit:
            VPMM_MCUEnableProc_flg = FALSE;
            (default) -> (junction 704) : {
                | VPMM_TimeMCUEnable_s = 0;
                | }
            MCUEnable -> (junction 704)
            (junction 704) -> (junction 705) : {
                | VPMM_VCUMCUEn_flg = TRUE;
                | }
            (junction 705) -> (junction 706) [order 1] : [VINP_MCUIGBTEnFbk_flg == TRUE]
            (junction 705) -> (junction 707) [order 2] : {
                | VPMM_TimeMCUEnable_s += task_time_s;
                | }
            (junction 706) -> (junction 708) : {
                | VPMM_MCUEnableProc_flg = FALSE;
                | VPMM_MCUEnableCompleted_flg = TRUE;
                | }
            (junction 708) -> (junction 707)
          (default) -> MCUPrechrg
          MCUPrechrg -> MCUEnable [order 1] : [VPMM_MCUPrechrgCompleted_flg]
        state PDU [parallel]
          settings: executionOrder=2
          state DCDC
            en:
            VPMM_DCDCEnableCompleted_flg = FALSE;
            VPMM_PowerUpState_enum = ENUM_PUSTATE_DCDCENABLE;
            VPMM_DCDCEnableProc_flg = TRUE;
            exit:
            VPMM_DCDCEnableProc_flg = FALSE;
            (default) -> (junction 903) : {
                | VPMM_TimeDCDCEnable_s = 0;
                | }
            DCDC -> (junction 903) [order 1]
            (junction 903) -> (junction 904) : {
                | VPMM_PMMDCDCEnableDem_flg = TRUE;
                | }
            (junction 904) -> (junction 905) [order 1] : [VINP_DCDCEnableStatus_enum == ENUM_DCDCENABLESTS_RUN]
            (junction 904) -> (junction 906) [order 2] : {
                | VPMM_TimeDCDCEnable_s += task_time_s;
                | }
            (junction 905) -> (junction 907) : {
                | VPMM_DCDCEnableCompleted_flg = TRUE;
                | }
            (junction 907) -> (junction 906)
          state EHPS
            en:
            VPMM_PowerUpState_enum = ENUM_PUSTATE_EHPSENABLE;
            VPMM_EHPSEnableProc_flg = TRUE;
            VPMM_TimeEHPSEnable_s = 0;
            VPMM_TimeEHPSIni_s = 0;
            VPMM_PMMEHPSDemSpd_rpm = 0;
            exit:
            VPMM_EHPSEnableProc_flg = FALSE;
            VPMM_PMMEHPSEnableDem_flg = FALSE;
            VPMM_PMMEHPSDemSpd_rpm = 0;
            (default) -> (junction 1355) : {
                | VPMM_PMMEHPSEnableDem_flg = TRUE;
                | }
            EHPS -> (junction 1355) [order 2]
            (junction 1355) -> (junction 1356) [order 1] : [VINP_EHPSEnableStatus_enum == ENUM_EHPSENABLESTS_RUN]
            EHPS -> (junction 1356) [order 1] : [VPMM_EHPSEnableCompleted_flg == TRUE]
            (junction 1355) -> (junction 1357) [order 2] : {
                | VPMM_TimeEHPSEnable_s += task_time_s;
                | }
            (junction 1356) -> (junction 1366) : {
                | VPMM_EHPSEnableCompleted_flg = TRUE;
                | VPMM_PMMEHPSDemSpd_rpm = KPMM_EHPSSpdDem_rpm;
                | }
            (junction 1366) -> (junction 1368) [order 1] : [VPMM_EHPSIniReady_flg == TRUE]
            (junction 1366) -> (junction 1358) [order 2] : {
                | VPMM_TimeEHPSIni_s += task_time_s;
                | }
            (junction 1368) -> (junction 1370) : {
                | VPMM_EHPSIniFinish_flg = TRUE;
                | }
            (junction 1358) -> (junction 1357)
            (junction 1370) -> (junction 1358)
          state EAC
            en:
            VPMM_PowerUpState_enum = ENUM_PUSTATE_EACPRESCHECK;
            VPMM_CACPresReadyProc_flg = TRUE;
            VPMM_TimeEACEnable_s = 0;
            VPMM_TimeWaitAirPress_s = 0;
            exit:
            VPMM_PMMEACEnableDem_flg = FALSE;
            VPMM_CACPresReadyProc_flg = FALSE;
            (default) -> (junction 1377) : {
                | VPMM_PMMEACEnableDem_flg = TRUE;
                | }
            EAC -> (junction 1377) [order 2]
            (junction 1377) -> (junction 1378) [order 1] : [VINP_EACEnSta_enum == ENUM_CACENABLESTS_RUN]
            EAC -> (junction 1378) [order 1] : [VPMM_EACEnableCompleted_flg]
            (junction 1377) -> (junction 1381) [order 2] : {
                | VPMM_TimeEACEnable_s += task_time_s;
                | }
            (junction 1378) -> (junction 1420) : {
                | VPMM_EACEnableCompleted_flg = TRUE;
                | VPMM_PMMEACEnableDem_flg = FALSE;
                | }
            (junction 1420) -> (junction 1422) [order 1] : [VACC_CACPresReady_flg]
            (junction 1420) -> (junction 1382) [order 2] : {
                | VPMM_TimeWaitAirPress_s += task_time_s;
                | }
            (junction 1422) -> (junction 1424) : {
                | VPMM_AirPressReady_flg = TRUE;
                | }
            (junction 1382) -> (junction 1381)
            (junction 1424) -> (junction 1382)
          (default) -> DCDC
          DCDC -> EHPS [order 1] : [VPMM_DCDCEnableCompleted_flg]
          EHPS -> EAC [order 1] : [VPMM_EHPSIniFinish_flg]
      state FindFaultRoot2
        en:
        VPMM_PDULoadPUFault_enum = ENUM_PUFAULT_NOFAULT;
        (default) -> (junction 809)
        (junction 809) -> (junction 810) [order 1] : [VPMM_PDUEACRlySta_enum ~= ENUM_CACRLYSTS_CLOSED]
        (junction 809) -> (junction 811) [order 2]
        (junction 810) -> (junction 818) : {
            | VPMM_PDULoadPUFault_enum = ENUM_PUFAULT_CACRLYUPFAIL;
            | }
        (junction 811) -> (junction 812) [order 1] : [VPMM_PDUEHPSRlySta_enum ~= ENUM_EHPSRLYSTS_CLOSED]
        (junction 811) -> (junction 813) [order 2]
        (junction 812) -> (junction 817) : {
            | VPMM_PDULoadPUFault_enum = ENUM_PUFAULT_EHPSRLYUPFAIL;
            | }
        (junction 813) -> (junction 814) [order 1] : [VINP_PDUACRlySta_enum ~= ENUM_PDUACRLYSTA_CLOSE]
        (junction 813) -> (junction 815) [order 2]
        (junction 814) -> (junction 816) : {
            | VPMM_PDULoadPUFault_enum = ENUM_PUFAULT_ACMAINRLYUPFAIL;
            | }
        (junction 816) -> (junction 815)
        (junction 817) -> (junction 816)
        (junction 818) -> (junction 817)
      state FindFaultRoot1
        en:
        (default) -> (junction 764)
        (junction 764) -> (junction 765) [order 1] : [(VPMM_TimeEHPSEnable_s > KPMM_EHPSENTimeout_s) || ...
            |  (VPMM_TimeEHPSIni_s > KPMM_EHPSIniTimeout_s)]
        (junction 764) -> (junction 766) [order 2] : {
            | VPMM_PowerUpFault_enum = ENUM_PUFAULT_AIRPRESS;
            | }
        (junction 765) -> (junction 767) : {
            | VPMM_PowerUpFault_enum = ENUM_PUFAULT_EHPSENABLEFAIL;
            | }
        (junction 767) -> (junction 766)
      state HVPwrReady
        en:
        VPMM_PowerUpState_enum = ENUM_PUSTATE_COMPLETED;
        VPMM_PowerUpComplete_flg = TRUE;
        VPMM_HVSysReady_enum = ENUM_HVSYSREADY_READY;
      state HVPwrFail
        en:
        VPMM_HVPwrFail_flg = TRUE;
      (default) -> BattPackPowerup
      BattPackPowerup -> (junction 743) [order 1] : [(VPMM_TimeBattPU_s > KPMM_BattUpFailtime_s) ||...
          | (VINP_BMSHVSts_enum == ENUM_BMSHVSTS_FAILTOHVON) ]
      (junction 743) -> HVPwrFail : {
          | VPMM_PowerUpFault_enum = ENUM_PUFAULT_BATTUPFAIL;
          | }
      BattPackPowerup -> Powerup.HVPwrUpProcess.DCDCRlyClosed [order 2] : [VPMM_BattPUCompleted_flg]
      Powerup.HVPwrUpProcess.DCDCRlyClosed -> (junction 744) [order 1] : [(VPMM_TimeDCDCRlyPU_s > KPMM_DCDCRlyUpFailtime_s) ||...
          | (VPMM_PDUDCDCRlySta_enum ==ENUM_DCDCRLYSTS_FAILTOCLOSE) ]
      (junction 744) -> HVPwrFail : {
          | VPMM_PowerUpFault_enum = ENUM_PUFAULT_DCDCRLYUPFAIL;
          | }
      Powerup.HVPwrUpProcess.DCDCRlyClosed -> PDULoadRlyClosed [order 2] : [VPMM_DCDCRlyUpCompleted_flg]
      PDULoadRlyClosed -> (junction 745) [order 1] : [(VPMM_TimePDULoadRlyPU_s > KPMM_PDULoadRlyPUFailtime_s) ||...
          |  (VPMM_PDUEACRlySta_enum == ENUM_CACRLYSTS_FAILTOCLOSE) ||...
          |  (VPMM_PDUEHPSRlySta_enum == ENUM_EHPSRLYSTS_FAILTOCLOSE) ||...
          |  (VINP_PDUACRlySta_enum== ENUM_PDUACRLYSTA_CLOSEFAILURE)]
      (junction 745) -> FindFaultRoot2
      PDULoadRlyClosed -> HVPwrEnable [order 2] : [VPMM_PDURelayPUReady_flg]
      HVPwrEnable -> (junction 746) [order 1] : [(VPMM_TimeMCUPrechrgRlyPU_s > KPMM_MCUPrechrgFailtime_s) ||...
          |  (VINP_MCUHVLoopSts_enum == ENUM_MCUHVLOOPSTS_FAILED) || ...
          |  (VINP_MCUFailGrade_enum ~= ZERO_INT)]
      (junction 746) -> HVPwrFail : {
          | VPMM_PowerUpFault_enum = ENUM_PUFAULT_MCUPRECHRGFAIL;
          | }
      HVPwrEnable -> (junction 747) [order 2] : [VPMM_TimeMCUEnable_s > KPMM_MCUEnableFailtime_s]
      (junction 747) -> HVPwrFail : {
          | VPMM_PowerUpFault_enum = ENUM_PUFAULT_MCUENABLEFAIL;
          | }
      HVPwrEnable -> (junction 748) [order 3] : [(VPMM_TimeDCDCEnable_s > KPMM_DCDCEnableFailtime_s) ||...
          | (VINP_DCDCEnableStatus_enum == ENUM_DCDCENABLESTS_FAULT)]
      FindFaultRoot2 -> HVPwrFail : {
          | VPMM_PowerUpFault_enum = VPMM_PDULoadPUFault_enum;
          | }
      (junction 748) -> HVPwrFail : {VPMM_PowerUpFault_enum = ENUM_PUFAULT_DCDCENABLEFAIL}
      HVPwrEnable -> (junction 749) [order 4] : [(VPMM_TimeEHPSEnable_s > KPMM_EHPSENTimeout_s) || ...
          |  (VPMM_TimeEHPSIni_s > KPMM_EHPSIniTimeout_s) || ...
          |  (VPMM_TimeEACEnable_s > KPMM_EACENTimeout_s) || ...
          |  (VPMM_TimeWaitAirPress_s > KPMM_WaitAirPressTimeout_s)]
      (junction 749) -> FindFaultRoot1
      HVPwrEnable -> HVPwrReady [order 5] : [VPMM_AirPressReady_flg && VPMM_MCUEnableCompleted_flg ]
      FindFaultRoot1 -> HVPwrFail
    state Timeout
      en:
      VPMM_PowerUpState_enum = ENUM_PUSTATE_POWERUPFAIL;
      VPMM_BattHVDem_enum = ENUM_BATTHVDEM_POWEROFF;
      VPMM_MCUHVLoopDem_enum = ENUM_MCUHVLOOP_POWEROFF;
      VPMM_PMMDCDCEnableDem_flg = FALSE;
      VPMM_DCDCRlyDem_enum = ENUM_DCDCRLYDEM_OPEN;
      VPMM_EHPSRlyDem_enum = ENUM_EHPSRLYDEM_OPEN;
      VPMM_CACRlyDem_enum = ENUM_CACRLYDEM_OPEN;
      VPMM_ACHVLoopDem_enum = ENUM_ACHVLOOP_POWEROFF;
      VPMM_VCUMCUEn_flg = FALSE;
      VPMM_PowerUpFail_flg = TRUE;
    (default) -> Powerup.Initialize
    Powerup.Initialize -> AlcLockcheck
    AlcLockcheck -> (junction 1343) [order 1] : [(VPMM_TimeAlcLockCheck_s > KPMM_AlcLockCheckFailtime_s)]
    (junction 1343) -> Timeout : {
        | VPMM_PowerUpFault_enum = ENUM_PUFAULT_ALINTERLOCK;
        | }
    AlcLockcheck -> HVRlycheck [order 2] : [VPMM_AlcLockCheckCompleted_flg]
    HVRlycheck -> (junction 877) [order 1] : [(VPMM_TimeHVRlyCheck_s > KPMM_HVRlyCheckFailtime_s)]
    (junction 877) -> Timeout : {
        | VPMM_PowerUpFault_enum = ENUM_PUFAULT_HVRLYCHKFAIL;
        | }
    HVRlycheck -> HVPwrUpProcess [order 2] : [VPMM_HVRlyCheckCompleted_flg]
    HVPwrUpProcess -> Timeout : [VPMM_HVPwrFail_flg]
  state Charge
    en:
    VPMM_SysPowerMode_enum = ENUM_PMMMODE_CHARGE;
    VPMM_ChrgIntoPwrdown_flg = FALSE;
    VPMM_PowerUpInhibit_flg = TRUE;
    VPMM_ChrgPowerUpFail_flg = FALSE;
    VPMM_HVRlyCheckCompleted_flg = FALSE;
    VPMM_ChrgPowerUpFail_flg = FALSE;
    VPMM_BattPUCompleted_flg = FALSE;
    VPMM_DCDCRlyUpCompleted_flg = FALSE;
    VPMM_ACMainRlyUpCompleted_flg = FALSE;
    VPMM_DCDCEnableCompleted_flg = FALSE;
    VPMM_CheckChrgStaFail_flg = FALSE;
    VPMM_CheckChrgSta_flg = FALSE;
    VPMM_DCDCNotEnaInChrg_flg =FALSE;
    VPMM_ChrgFinishComplete_flg = FALSE;
    VPMM_BattHVDem_enum = ENUM_BATTHVDEM_POWEROFF;
    VPMM_DCDCRlyDem_enum = ENUM_DCDCRLYDEM_OPEN;
    VPMM_EHPSRlyDem_enum = ENUM_EHPSRLYDEM_OPEN;
    VPMM_CACRlyDem_enum = ENUM_CACRLYDEM_OPEN;
    VPMM_MCUHVLoopDem_enum = ENUM_MCUHVLOOP_POWEROFF;
    VPMM_ACHVLoopDem_enum = ENUM_ACHVLOOP_POWEROFF;
    state HVRlyCheck
      en:
      VPMM_ChrgState_enum = ENUM_CHRGSTATE_CHECKHVRLYOPEN;
      VPMM_HVRlyCheckCompleted_flg = FALSE;
      VPMM_ChrgPowerUpFail_flg = FALSE;
      VPMM_TimeHVRlyCheck_s = 0;
      (default) -> (junction 697) : {
          | VPMM_HVRlyCheckCompleted_flg = FALSE;
          | VPMM_BattHVDem_enum = ENUM_BATTHVDEM_POWEROFF;
          | VPMM_DCDCRlyDem_enum = ENUM_DCDCRLYDEM_OPEN;
          | VPMM_EHPSRlyDem_enum = ENUM_EHPSRLYDEM_OPEN;
          | VPMM_CACRlyDem_enum = ENUM_CACRLYDEM_OPEN;
          | VPMM_MCUHVLoopDem_enum = ENUM_MCUHVLOOP_POWEROFF;
          | VPMM_ACHVLoopDem_enum = ENUM_ACHVLOOP_POWEROFF;
          | }
      HVRlyCheck -> (junction 697) [order 1]
      (junction 697) -> (junction 698) [order 1] : [VPMM_RlyOpenCheck_flg]
      (junction 697) -> (junction 699) [order 2]
      (junction 698) -> (junction 703) : {
          | VPMM_HVRlyCheckCompleted_flg = TRUE;
          | }
      (junction 699) -> (junction 700) [order 1] : [VPMM_TimeHVRlyCheck_s > KPMM_HVRlyCheckFailtime_s]
      (junction 699) -> (junction 701) [order 2] : {
          | VPMM_TimeHVRlyCheck_s += task_time_s;
          | }
      (junction 700) -> (junction 702) : {
          | VPMM_ChrgFault_enum = ENUM_CHRGFAULT_RLYCHKFAIL;
          | VPMM_ChrgPowerUpFail_flg = TRUE;
          | }
      (junction 702) -> (junction 701)
      (junction 703) -> (junction 702)
    state BCUPowerUp
      en:
      VPMM_ChrgState_enum = ENUM_CHRGSTATE_BCUNEGRLYCLOSED;
      VPMM_BattPUCompleted_flg = FALSE;
      VPMM_ChrgPowerUpFail_flg = FALSE;
      VPMM_TimeBattPU_s = 0;
      (default) -> (junction 652) : {
          | VPMM_BattHVDem_enum = ENUM_BATTHVDEM_POWERON;
          | }
      BCUPowerUp -> (junction 652) [order 1]
      (junction 652) -> (junction 653) [order 1] : [VINP_BMSHVSts_enum ==ENUM_BMSHVSTS_HVCLOSED]
      (junction 652) -> (junction 654) [order 2]
      (junction 653) -> (junction 658) : {
          | VPMM_BattPUCompleted_flg = TRUE;
          | }
      (junction 654) -> (junction 655) [order 1] : [(VPMM_TimeBattPU_s > KPMM_BattUpFailtime_s) ||...
          |  (VINP_BMSHVSts_enum == ENUM_BMSHVSTS_FAILTOHVON)]
      (junction 654) -> (junction 656) [order 2] : {
          | VPMM_TimeBattPU_s += task_time_s;
          | }
      (junction 655) -> (junction 657) : {
          | VPMM_ChrgFault_enum = ENUM_CHRGFAULT_BCUNEGFAIL;
          | VPMM_ChrgPowerUpFail_flg = TRUE;
          | }
      (junction 657) -> (junction 656)
      (junction 658) -> (junction 657)
    state DCDCRlyClosed
      en:
      VPMM_ChrgState_enum = ENUM_CHRGSTATE_DCDCRLYCLOSED;
      VPMM_DCDCRlyUpCompleted_flg = FALSE;
      VPMM_ChrgPowerUpFail_flg = FALSE;
      VPMM_TimeDCDCRlyDemDelay_s = 0;
      VPMM_TimeDCDCRlyPU_s = 0;
      (default) -> (junction 614)
      Charge.DCDCRlyClosed -> (junction 614) [order 1]
      (junction 614) -> (junction 615) [order 1] : [VPMM_TimeDCDCRlyDemDelay_s > KPMM_DCDCRlyDemDelayTime_s]
      (junction 614) -> (junction 620) [order 2] : {
          | VPMM_TimeDCDCRlyDemDelay_s += task_time_s;
          | }
      (junction 615) -> (junction 616) : {
          | VPMM_DCDCRlyDem_enum = ENUM_DCDCRLYDEM_CLOSE;
          | }
      (junction 616) -> (junction 617) [order 1] : [VPMM_PDUDCDCRlySta_enum == ENUM_DCDCRLYSTS_CLOSED]
      (junction 616) -> (junction 618) [order 2]
      (junction 617) -> (junction 623) : {
          | VPMM_DCDCRlyUpCompleted_flg = TRUE;
          | }
      (junction 618) -> (junction 619) [order 1] : [(VPMM_TimeDCDCRlyPU_s > KPMM_DCDCRlyUpFailtime_s) ||...
          | (VPMM_PDUDCDCRlySta_enum ==ENUM_DCDCRLYSTS_FAILTOCLOSE) ]
      (junction 618) -> (junction 621) [order 2] : {
          | VPMM_TimeDCDCRlyPU_s += task_time_s;
          | }
      (junction 619) -> (junction 622) : {
          | VPMM_ChrgFault_enum = ENUM_CHRGFAULT_DCDCRLYFAIL;
          | VPMM_ChrgPowerUpFail_flg = TRUE;
          | }
      (junction 620) -> (junction 621)
      (junction 622) -> (junction 621)
      (junction 623) -> (junction 622)
    state ACHVPowerUp
      en:
      VPMM_ChrgState_enum = ENUM_CHRGSTATE_ACRLYCLOSED;
      VPMM_ACMainRlyUpCompleted_flg = FALSE;
      VPMM_ChrgPowerUpFail_flg = FALSE;
      VPMM_TimeACMainRlyPU_s = 0;
      (default) -> (junction 690) : {
          | VPMM_ACHVLoopDem_enum = ENUM_ACHVLOOP_POWERON;
          | }
      ACHVPowerUp -> (junction 690) [order 1]
      (junction 690) -> (junction 691) [order 1] : [VINP_PDUACRlySta_enum== ENUM_PDUACRLYSTA_CLOSE]
      (junction 690) -> (junction 692) [order 2]
      (junction 691) -> (junction 696) : {
          | VPMM_ACMainRlyUpCompleted_flg = TRUE;
          | }
      (junction 692) -> (junction 693) [order 1] : [(VPMM_TimeACMainRlyPU_s > KPMM_ACMainRlyUpFailtime_s) ||...
          |  (VINP_PDUACRlySta_enum== ENUM_PDUACRLYSTA_CLOSEFAILURE) ]
      (junction 692) -> (junction 694) [order 2] : {
          | VPMM_TimeACMainRlyPU_s += task_time_s;
          | }
      (junction 693) -> (junction 695) : {
          | VPMM_ChrgFault_enum = ENUM_CHRGFAULT_ACRLYFAIL;
          | VPMM_ChrgPowerUpFail_flg = TRUE;
          | }
      (junction 695) -> (junction 694)
      (junction 696) -> (junction 695)
    state DCDCEnable
      en:
      VPMM_ChrgState_enum = ENUM_CHRGSTATE_DCDCENABLE;
      VPMM_DCDCEnableCompleted_flg = FALSE;
      VPMM_ChrgPowerUpFail_flg = FALSE;
      VPMM_TimeDCDCEnable_s = 0;
      (default) -> (junction 624) : {
          | VPMM_PMMDCDCEnableDem_flg = TRUE;
          | }
      DCDCEnable -> (junction 624) [order 1]
      (junction 624) -> (junction 625) [order 1] : [VINP_DCDCEnableStatus_enum == ENUM_DCDCENABLESTS_RUN]
      (junction 624) -> (junction 626) [order 2]
      (junction 625) -> (junction 630) : {
          | VPMM_DCDCEnableCompleted_flg = TRUE;
          | }
      (junction 626) -> (junction 627) [order 1] : [(VPMM_TimeDCDCEnable_s > KPMM_DCDCEnableFailtime_s) ||...
          | (VINP_DCDCEnableStatus_enum == ENUM_DCDCENABLESTS_FAULT)]
      (junction 626) -> (junction 628) [order 2] : {
          | VPMM_TimeDCDCEnable_s += task_time_s;
          | }
      (junction 627) -> (junction 629) : {
          | VPMM_ChrgFault_enum = ENUM_CHRGFAULT_DCDCENABLE;
          | VPMM_ChrgPowerUpFail_flg = TRUE;
          | }
      (junction 629) -> (junction 628)
      (junction 630) -> (junction 629)
    state CheckChrgSta
      en:
      VPMM_ChrgState_enum = ENUM_CHRGSTATE_CHKCHRGSTA;
      VPMM_CheckChrgSta_flg = FALSE;
      VPMM_CheckChrgStaFail_flg = FALSE;
      VPMM_TimeBCUGetChrg_s = 0;
      (default) -> (junction 641)
      CheckChrgSta -> (junction 641) [order 1]
      (junction 641) -> (junction 642) [order 1] : [VINP_BMSChrgStatus_enum == ENUM_BMSCHRGSTS_CHARGING]
      (junction 641) -> (junction 643) [order 2]
      (junction 642) -> (junction 647) : {
          | VPMM_CheckChrgSta_flg = TRUE;
          | }
      (junction 643) -> (junction 644) [order 1] : [VPMM_TimeBCUGetChrg_s > KPMM_BCUGetChrgTO_s]
      (junction 643) -> (junction 645) [order 2] : {
          | VPMM_TimeBCUGetChrg_s += task_time_s;
          | }
      (junction 644) -> (junction 646) : {
          | VPMM_ChrgFault_enum = ENUM_CHRGFAULT_BCUTIMEOUT;
          | VPMM_CheckChrgStaFail_flg = TRUE;
          | }
      (junction 646) -> (junction 645)
      (junction 647) -> (junction 646)
    state ChargeFinish
      en:
      VPMM_ChrgState_enum = ENUM_CHRGSTATE_FINISH;
      VPMM_ChrgIntoPwrdown_flg = FALSE;
      VPMM_TimeChrgIntoPwrdownWait_s = 0
      (default) -> (junction 631)
      ChargeFinish -> (junction 631)
      (junction 631) -> (junction 632) [order 1] : [VPMM_TimeChrgIntoPwrdownWait_s > KPMM_ChrgIntoPwrdownWait_s]
      (junction 631) -> (junction 633) [order 2] : {
          | VPMM_TimeChrgIntoPwrdownWait_s += task_time_s;
          | }
      (junction 632) -> (junction 634) : {
          | VPMM_ChrgIntoPwrdown_flg = TRUE;
          | }
      (junction 634) -> (junction 633)
    state Charging
      en:
      VPMM_ChrgState_enum = ENUM_CHRGSTATE_CHARGING;
      VPMM_ChrgFinishComplete_flg = FALSE;
      VPMM_DCDCNotEnaInChrg_flg = FALSE;
      VPMM_IGNRlyClose_flg = FALSE;
      VPMM_SSBrisevent_flg = FALSE;
      VPMM_ChrgIGNTrig_flg = FALSE;
      VPMM_ButtonHoldtime_cnt = 0;
      VPMM_TimeDCDCChrgNotEna_s = 0;
      VPMM_TimeChrgIntoPwrdownWait_s =0;
      state Charging IGNrly trig [group]
        (junction 780) -> (junction 781) [order 1] : [VPMM_SSBrisdetect_flg]
        (junction 780) -> (junction 782) [order 2]
        (junction 781) -> (junction 783) : {VPMM_SSBrisevent_flg = TRUE}
        (junction 783) -> (junction 782)
        (junction 782) -> (junction 784)
        (junction 784) -> (junction 785) [order 1] : [VINP_PushButton_flg &&...
            | VPMM_SSBrisevent_flg]
        (junction 785) -> (junction 786) [order 1] : [VPMM_ButtonHoldtime_cnt > KPMM_ButtonHoldlimit_cnt]
        (junction 784) -> (junction 787) [order 2] : {
            | VPMM_ButtonHoldtime_cnt = 0;
            | VPMM_ChrgIGNTrig_flg = FALSE;
            | VPMM_SSBrisevent_flg = FALSE;
            | }
        (junction 785) -> (junction 788) [order 2] : {VPMM_ButtonHoldtime_cnt += 1}
        (junction 786) -> (junction 789) : {VPMM_ChrgIGNTrig_flg = TRUE}
        (junction 788) -> (junction 787)
        (junction 789) -> (junction 788)
        (junction 787) -> (junction 791)
        (junction 791) -> (junction 790) [order 2] : [
            | VPMM_ChrgIGNTrig_flg && VPMM_IGNRlyClose_flg
            | ]
        (junction 791) -> (junction 792) [order 1] : [
            | VPMM_ChrgIGNTrig_flg && !VPMM_IGNRlyClose_flg
            | ]
        (junction 790) -> (junction 794) : {
            | VPMM_IGNRlyClose_flg = FALSE;
            | VPMM_SSBrisevent_flg = FALSE;
            | VPMM_ChrgIGNTrig_flg = FALSE;
            | VPMM_ButtonHoldtime_cnt = 0;
            | }
        (junction 791) -> (junction 795) [order 3]
        (junction 792) -> (junction 793) : {
            | VPMM_IGNRlyClose_flg = TRUE;
            | VPMM_SSBrisevent_flg = FALSE;
            | VPMM_ChrgIGNTrig_flg = FALSE;
            | VPMM_ButtonHoldtime_cnt = 0;
            | }
        (junction 794) -> (junction 795)
        (junction 793) -> (junction 795)
      (default) -> (junction 713)
      (junction 713) -> (junction 714) [order 1] : [VINP_DCDCEnableStatus_enum ~= ENUM_DCDCENABLESTS_RUN]
      Charging -> (junction 713) [order 1]
      (junction 714) -> (junction 717) : {
          | VPMM_TimeDCDCChrgNotEna_s += task_time_s;
          | }
      (junction 713) -> (junction 715) [order 2] : {
          | VPMM_TimeDCDCChrgNotEna_s =0;
          | }
      (junction 715) -> (junction 716) [order 1] : [((VINP_BMSChrgStatus_enum == ENUM_BMSCHRGSTS_FINISH) || ...
          |  (VINP_ChargeWakeup_flg == FALSE) || ...
          |  (VINP_DCChrgConnectSts_enum ~= ENUM_PLUGINSTS_PLUGIN))]
      (junction 715) -> (junction 780) [order 2] : {
          | VPMM_TimeChrgIntoPwrdownWait_s =0;
          | }
      (junction 716) -> (junction 1313)
      (junction 1313) -> (junction 1315) [order 1] : [VPMM_TimeChrgIntoPwrdownWait_s > KPMM_ChrgIntoPwrdownWait_s]
      (junction 1313) -> (junction 1319) [order 2] : {
          | VPMM_TimeChrgIntoPwrdownWait_s += task_time_s;
          | }
      (junction 1315) -> (junction 1317) : {
          | VPMM_ChrgFinishComplete_flg = TRUE;
          | }
      (junction 1317) -> (junction 1319)
      (junction 1319) -> (junction 720)
      (junction 717) -> (junction 718) [order 1] : [VPMM_TimeDCDCChrgNotEna_s > KPMM_DCDCChrgFailtime_s]
      (junction 717) -> (junction 721) [order 2]
      (junction 718) -> (junction 722) : {
          | VPMM_DCDCNotEnaInChrg_flg = TRUE;
          | }
      (junction 795) -> (junction 719)
      (junction 722) -> (junction 721)
      (junction 721) -> (junction 720)
      (junction 719) -> (junction 720)
    state ChargeError
      en:
      VPMM_ChrgState_enum = ENUM_CHRGSTATE_ERROR;
      VPMM_TimeChrgIntoPwrdownWait_s = 0;
      VPMM_ChrgIntoPwrdown_flg = FALSE;
      VPMM_BattHVDem_enum = ENUM_BATTHVDEM_POWEROFF;
      VPMM_MCUHVLoopDem_enum = ENUM_MCUHVLOOP_POWEROFF;
      VPMM_PMMDCDCEnableDem_flg = FALSE;
      VPMM_DCDCRlyDem_enum = ENUM_DCDCRLYDEM_OPEN;
      VPMM_EHPSRlyDem_enum = ENUM_EHPSRLYDEM_OPEN;
      VPMM_CACRlyDem_enum = ENUM_CACRLYDEM_OPEN;
      VPMM_ACHVLoopDem_enum = ENUM_ACHVLOOP_POWEROFF;
      VPMM_VCUMCUEn_flg = FALSE;
      VPMM_ChrgPEUFail_flg = FALSE;
      VPMM_ChrgBCUHVFail_flg = FALSE;
      (default) -> (junction 659)
      ChargeError -> (junction 659)
      (junction 659) -> (junction 660) [order 1] : [!VPMM_HVFailureChkPass_flg]
      (junction 659) -> (junction 661) [order 2]
      (junction 660) -> (junction 667)
      (junction 661) -> (junction 662) [order 1] : [VPMM_DCDCNotEnaInChrg_flg]
      (junction 661) -> (junction 671) [order 2]
      (junction 662) -> (junction 672) : {
          | VPMM_ChrgFault_enum = ENUM_CHRGFAULT_DCDCENABLE;
          | }
      (junction 667) -> (junction 668) [order 1] : [(VINP_PEUSelfChkSts_enum ~= ENUM_PEUSELFCHKSTS_NOFAULT)&& ...
          |   !VPMM_ChrgPEUFail_flg]
      (junction 667) -> (junction 669) [order 2]
      (junction 668) -> (junction 675) : {
          | VPMM_ChrgPEUFail_flg = TRUE;
          | VPMM_ChrgFault_enum = ENUM_CHRGFAULT_PDUHVFAIL;
          | }
      (junction 669) -> (junction 670) [order 1] : [(VINP_HVPwrOffReq_enum == ENUM_HVPWROFFREQ_POWEROFF) && ...
          |   !VPMM_ChrgBCUHVFail_flg]
      (junction 669) -> (junction 673) [order 2]
      (junction 670) -> (junction 674) : {
          | VPMM_ChrgBCUHVFail_flg = TRUE;
          | VPMM_ChrgFault_enum = ENUM_CHRGFAULT_BCUHVFAIL;
          | }
      (junction 672) -> (junction 671)
      (junction 673) -> (junction 672)
      (junction 674) -> (junction 673)
      (junction 675) -> (junction 674)
      (junction 671) -> (junction 678) : {
          | VPMM_TimeChrgIntoPwrdownWait_s += task_time_s;
          | }
      (junction 678) -> (junction 679) [order 1] : [VPMM_HVILEmergencyStop_flg]
      (junction 678) -> (junction 680) [order 2]
      (junction 679) -> (junction 681) : {
          | VPMM_ChrgFault_enum = ENUM_CHRGFAULT_HVILFAIL;
          | }
      (junction 680) -> (junction 681) [order 1] : [VPMM_TimeChrgIntoPwrdownWait_s > KPMM_ChrgIntoPwrdownWait_s]
      (junction 680) -> (junction 682) [order 2]
      (junction 681) -> (junction 683) : {
          | VPMM_ChrgIntoPwrdown_flg = TRUE;
          | }
      (junction 683) -> (junction 682)
    (default) -> HVRlyCheck
    HVRlyCheck -> (junction 635) [order 1] : [VPMM_ChrgPowerUpFail_flg || !VPMM_HVFailureChkPass_flg]
    (junction 635) -> (junction 636)
    HVRlyCheck -> BCUPowerUp [order 2] : [VPMM_HVRlyCheckCompleted_flg]
    BCUPowerUp -> (junction 636) [order 1] : [VPMM_ChrgPowerUpFail_flg || !VPMM_HVFailureChkPass_flg]
    (junction 636) -> (junction 637)
    BCUPowerUp -> Charge.DCDCRlyClosed [order 2] : [VPMM_BattPUCompleted_flg]
    Charge.DCDCRlyClosed -> (junction 637) [order 1] : [VPMM_ChrgPowerUpFail_flg || !VPMM_HVFailureChkPass_flg]
    (junction 637) -> (junction 638)
    Charge.DCDCRlyClosed -> ACHVPowerUp [order 2] : [VPMM_DCDCRlyUpCompleted_flg]
    ACHVPowerUp -> (junction 638) [order 1] : [VPMM_ChrgPowerUpFail_flg || !VPMM_HVFailureChkPass_flg]
    (junction 638) -> (junction 639)
    ACHVPowerUp -> DCDCEnable [order 2] : [VPMM_ACMainRlyUpCompleted_flg]
    DCDCEnable -> (junction 639) [order 1] : [VPMM_ChrgPowerUpFail_flg || !VPMM_HVFailureChkPass_flg]
    (junction 639) -> (junction 640)
    DCDCEnable -> CheckChrgSta [order 2] : [VPMM_DCDCEnableCompleted_flg]
    CheckChrgSta -> (junction 640) [order 1] : [VPMM_CheckChrgStaFail_flg || !VPMM_HVFailureChkPass_flg]
    (junction 640) -> ChargeError
    CheckChrgSta -> Charging [order 2] : [VPMM_CheckChrgSta_flg]
    Charging -> ChargeFinish [order 2] : [VPMM_ChrgFinishComplete_flg]
    Charging -> ChargeError [order 1] : [VPMM_DCDCNotEnaInChrg_flg || ...
        |  !VPMM_HVFailureChkPass_flg ]
  state AfterRun
    en:
    VPMM_SysPowerMode_enum = ENUM_PMMMODE_AFTERRUN;
    VPMM_NoAfterRunRequest_flg = FALSE;
    VPMM_ForceOffInAfterun_flg = FALSE;
    VPMM_AfterrunCompleted_flg = FALSE;
    state IGNRlyOpen
      en:
      VPMM_NoAfterRunRequest_flg = FALSE;
      (default) -> (junction 1474) : {
          | VPMM_TimeWaitForAfterrun_s = 0;
          | }
      IGNRlyOpen -> (junction 1474) [order 1]
      (junction 1474) -> (junction 1476) [order 1] : [VPSA_Keystatus_enum == ENUM_KEYSTATUS_OFF]
      (junction 1474) -> (junction 709) [order 2]
      (junction 1476) -> (junction 1478) : {
          | VPMM_IGNRlyClose_flg = TRUE;
          | }
      (junction 1478) -> (junction 709)
      (junction 709) -> (junction 1482)
      (junction 1482) -> (junction 710) [order 1] : [VPMM_TimeWaitForAfterrun_s > KPMM_WaitForAfterrunFail_s]
      (junction 1482) -> (junction 711) [order 2] : {
          | VPMM_TimeWaitForAfterrun_s += task_time_s;
          | }
      (junction 710) -> (junction 712) : {
          | VPMM_NoAfterRunRequest_flg = TRUE;
          | }
      (junction 712) -> (junction 711)
    state MCUAfterrun
      en:
      VPMM_ForceOffInAfterun_flg = FALSE;
      VPMM_ChrgIGNTrig_flg = FALSE;
      VPMM_SSBrisevent_flg = FALSE;
      VPMM_ButtonHoldtime_cnt = 0;
      (default) -> (junction 648) : {
          | VPMM_TimeForceOffInAfterrun_s = 0;
          | }
      (junction 648) -> (junction 649) [order 1] : [VPMM_TimeForceOffInAfterrun_s > KPMM_AfterrunTimeout_s ||...
          | VINP_VCUBattVol_v < KPMM_VoltForceOffInAfferun_v]
      MCUAfterrun -> (junction 648) [order 1]
      (junction 648) -> (junction 1436) [order 2] : {
          | VPMM_TimeForceOffInAfterrun_s += task_time_s;
          | }
      (junction 649) -> (junction 651) : {
          | VPMM_ForceOffInAfterun_flg = TRUE;
          | }
      (junction 1436) -> (junction 1432) [order 1] : [VPMM_SSBrisdetect_flg]
      (junction 1436) -> (junction 1438) [order 2]
      (junction 1432) -> (junction 1431) : {VPMM_SSBrisevent_flg = TRUE}
      (junction 1431) -> (junction 1438)
      (junction 1438) -> (junction 1450)
      (junction 1450) -> (junction 1440) [order 1] : [VINP_PushButton_flg &&...
          | VPMM_SSBrisevent_flg]
      (junction 1440) -> (junction 1441) [order 1] : [VPMM_ButtonHoldtime_cnt > KPMM_ButtonHoldlimit_cnt]
      (junction 1450) -> (junction 1452) [order 2] : {VPMM_ButtonHoldtime_cnt == 0}
      (junction 1440) -> (junction 1442) [order 2] : {VPMM_ButtonHoldtime_cnt += 1}
      (junction 1441) -> (junction 1443) : {VPMM_ChrgIGNTrig_flg = TRUE}
      (junction 1442) -> (junction 1452)
      (junction 1443) -> (junction 1442)
      (junction 1452) -> (junction 1459)
      (junction 1459) -> (junction 1454) [order 1] : [VPMM_ChrgIGNTrig_flg]
      (junction 1459) -> (junction 1461) [order 2]
      (junction 1454) -> (junction 1455) : {
          | VPMM_PowerUpInhibit_flg = FALSE;
          | VPMM_SSBrisevent_flg = FALSE;
          | VPMM_ChrgIGNTrig_flg = FALSE;
          | VPMM_ButtonHoldtime_cnt = 0;
          | }
      (junction 1455) -> (junction 1461)
      (junction 651) -> (junction 1455)
    state AfterrunCompleted
      en:
      VPMM_AfterrunCompleted_flg = TRUE;
    (default) -> IGNRlyOpen
    IGNRlyOpen -> MCUAfterrun [order 1] : [VINP_MCUAfterRunReq_flg ||...
        | VTHC_AfterrunningMode_flg]
    MCUAfterrun -> AfterrunCompleted [order 1] : [(!VINP_MCUAfterRunReq_flg && !VTHC_AfterrunningMode_flg) ||...
        |  VPMM_ForceOffInAfterun_flg]
    IGNRlyOpen -> (junction 684) [order 2]
    (junction 684) -> AfterrunCompleted : [VPMM_NoAfterRunRequest_flg]
  (default) -> Initialize
  Sleep -> Initialize : [KPSA_FakeWakeRESETRising_flg]
  Initialize -> Standby : [VPMM_Boot2Initialize_flg && VPMM_ChrgwakeDebon_cnt > KPMM_ChrgwakeDebon_cnt]
  Idle -> Sleep [order 1] : [VPMM_PwrOffCompleted_flg]
  (junction 915) -> Standby
  (junction 920) -> (junction 915)
  Standby -> (junction 916) [order 3] : [VPMM_Initialize2Charge_flg && VPMM_HVSelfChkCompleted4Chrg_flg]
  (junction 916) -> (junction 919)
  Standby -> Idle [order 1] : [(VPMM_Initialize2Idle_flg ||(VPMM_SysInitialTO_flg)) && VINP_ParkBrakeSW_flg]
  Standby -> (junction 917) [order 2] : [VPMM_HVSelfChkCompleted4PU_flg && VPMM_Initialize2PowerUp_flg]
  (junction 917) -> Powerup
  Drive -> Powerdown [order 1] : [VPMM_Drive2PowerDown_flg]
  Powerup -> Drive [order 2] : [VPMM_PowerUpComplete_flg]
  Powerup -> (junction 918) [order 1]
  (junction 918) -> Powerdown : [VPMM_PowerUp2PowerDown_flg ]
  Charge -> Powerdown : [VPMM_ChrgIntoPwrdown_flg || VPMM_Charge2PowerDown_flg ]
  (junction 919) -> Charge
  Powerdown -> AfterRun : [VPMM_PowerDownCompleted_flg]
  AfterRun -> (junction 920) [order 2] : [VPMM_AfterRun2Initialize_flg]
  AfterRun -> Idle [order 1] : [
      | ((VPMM_AfterrunCompleted_flg && ...
      | VPSA_Keystatus_enum == ENUM_KEYSTATUS_OFF) || ...
      | (VPMM_MCUSta2Lost_flg && ...
      | VPSA_Keystatus_enum == ENUM_KEYSTATUS_OFF) || ...
      | (VPMM_LVChrgFinished_flg || VPMM_LVChrgPreActFinished_flg))...
      | && VINP_ParkBrakeSW_flg
      | ]
  data: ENUM_EHPSENABLESTS_READY parameter; VACC_CACPresReady_flg input; VPSA_Keystatus_enum input; VPMM_RlyOpenCheck_flg input; VINP_BMSHVSts_enum input; VINP_DCChrgConnectSts_enum input; VPMM_PDUDCDCRlySta_enum input; VPMM_PDUEHPSRlySta_enum input; VPMM_PDUEACRlySta_enum input; VINP_MCUHVLoopSts_enum input; VINP_DCDCEnableStatus_enum input; VINP_EHPSEnableStatus_enum input; VINP_EACEnSta_enum input; VINP_MCUInVol_V input; VPMM_SysPowerMode_enum output; VPMM_PowerUpState_enum output uint8; VPMM_PowerDownState_enum output uint8; VPMM_ChrgState_enum output uint8; VPMM_PowerUpFault_enum output uint8; VPMM_PowerDownFault_enum output uint8; VPMM_ChrgFault_enum output uint8; VPMM_IRCRlyClose_flg output boolean; VPMM_IGNRlyClose_flg output boolean; VPMM_BattHVDem_enum output uint8; VPMM_DCDCRlyDem_enum output uint8; VPMM_CACRlyDem_enum output uint8; VPMM_MCUHVLoopDem_enum output uint8; VPMM_EHPSRlyDem_enum output uint8; VPMM_ACHVLoopDem_enum output uint8; VPMM_HVSysReady_enum output uint8; VPMM_DrivelineRelease_enum output uint8; VPMM_PMMDCDCEnableDem_flg output boolean; VINP_BMSChrgStatus_enum input; VINP_ChargeWakeup_flg input; VINP_HVPwrOffReq_enum input; VINP_MCUAfterRunReq_flg input; VINP_MCUIGBTEnFbk_flg input; KPMM_HVRlyCheckFailtime_s input; KPMM_BattUpFailtime_s input; KPMM_DCDCRlyUpFailtime_s input; KPMM_DCDCEnableFailtime_s input; KPMM_ACMainRlyUpFailtime_s input; KPMM_MCUPrechrgFailtime_s input; KPMM_BattDownFailtime_s input; KPMM_MCUDisChrgFailtime_s input; KPMM_DCDCChrgFailtime_s input; KPMM_TargetDchrgVolt_V input; VPMM_PowerUpInhibit_flg output boolean; VPMM_ACMainRlyUpCompleted_flg local boolean; VPMM_BattPDCompleted_flg local boolean; VPMM_BattPackPDFail_flg local boolean; VPMM_CACRlyUpCompleted_flg local boolean; VPMM_DCDCRlyUpCompleted_flg local boolean; VPMM_EHPSRlyUpCompleted_flg local boolean; VPMM_HVRlyCheckCompleted_flg local boolean; VPMM_HVSelfChkCompleted_flg local boolean; VPMM_HVSelfChkFail_flg local boolean; VPMM_MCUDisChrgCompleted_flg local boolean; VPMM_MainRlyOpenCompleted_flg local boolean; VPMM_PowerUpFail_flg local boolean; VPMM_TimeACMainRlyPU_s local single; VPMM_TimeBattPD_s local single; VPMM_TimeBattPU_s local single; VPMM_TimeDCDCEnable_s local single; VPMM_TimeDCDCRlyPU_s local single; VPMM_TimeHVRlyCheck_s local single; VPMM_TimeHVSelfChk_s local single; VPMM_TimeMCUDisChrg_s local single; VPMM_TimeMCUPrechrgRlyPU_s local single; ENUM_BATTHVDEM_POWEROFF parameter; ENUM_BATTHVDEM_POWERON parameter; ENUM_BMSCHRGSTS_FINISH parameter; ENUM_BMSHVSTS_FAILTOHVON parameter; ENUM_BMSHVSTS_HVCLOSED parameter; ENUM_BMSHVSTS_HVOPEN parameter; ENUM_CACENABLESTS_RUN parameter; ENUM_CACRLYDEM_CLOSE parameter; ENUM_CACRLYDEM_OPEN parameter; ENUM_CACRLYSTS_CLOSED parameter; ENUM_CACRLYSTS_FAILTOCLOSE parameter; ENUM_CACRLYSTS_OPEN parameter; ENUM_CHRGFAULT_NOFAULT parameter; ENUM_CHRGFAULT_RLYCHKFAIL parameter; ENUM_CHRGSTATE_CHARGING parameter; ENUM_CHRGSTATE_FINISH parameter; ENUM_DCDCENABLESTS_FAULT parameter; ENUM_DCDCENABLESTS_RUN parameter; ENUM_DCDCRLYDEM_CLOSE parameter; ENUM_DCDCRLYDEM_OPEN parameter; ENUM_DCDCRLYSTS_CLOSED parameter; ENUM_DCDCRLYSTS_FAILTOCLOSE parameter; ENUM_DCDCRLYSTS_OPEN parameter; ENUM_DRIVELINERELEASE_NOTRELEASE parameter; ENUM_DRIVELINERELEASE_RELEASE parameter; ENUM_EHPSENABLESTS_RUN parameter; ENUM_EHPSRLYDEM_CLOSE parameter; ENUM_EHPSRLYDEM_OPEN parameter; ENUM_EHPSRLYSTS_CLOSED parameter; ENUM_EHPSRLYSTS_FAILTOCLOSE parameter; ENUM_EHPSRLYSTS_OPEN parameter; ENUM_HVSYSREADY_NOTREADY parameter; ENUM_HVSYSREADY_READY parameter; ENUM_PDFAULT_MCUDISCHRG parameter; ENUM_PDFAULT_NOFAULT parameter; ENUM_PLUGINSTS_NOPLUGIN parameter; ENUM_PLUGINSTS_PLUGIN parameter; ENUM_PMMMODE_AFTERRUN parameter; ENUM_PMMMODE_CHARGE parameter; ENUM_PMMMODE_DRIVE parameter; ENUM_PMMMODE_POWERDOWN parameter; ENUM_PMMMODE_POWERUP parameter; ENUM_PUFAULT_ACMAINRLYUPFAIL parameter; ENUM_PUFAULT_BATTUPFAIL parameter; ENUM_PUFAULT_CACRLYUPFAIL parameter; ENUM_PUFAULT_DCDCENABLEFAIL parameter; ENUM_PUFAULT_DCDCRLYUPFAIL parameter; ENUM_PUFAULT_EHPSRLYUPFAIL parameter; ENUM_PUFAULT_MCUPRECHRGFAIL parameter; ENUM_PUFAULT_NOFAULT parameter; ENUM_PUSTATE_BCUPOSRLYCLOSED parameter; ENUM_PUSTATE_COMPLETED parameter; ENUM_PUSTATE_HVRLYCHECK parameter; ENUM_PUSTATE_INITIALIZE parameter; ENUM_PUSTATE_POWERUPFAIL parameter; FALSE parameter; TRUE parameter; VPMM_BattPUCompleted_flg local boolean; VPMM_PowerDownCompleted_flg output boolean; VPMM_PowerUpComplete_flg output boolean; VPMM_MCUPrechrgCompleted_flg local boolean; KPMM_TimeHVSelfChk4Chrg_s input; KPMM_SysInitialTO_s input; KPMM_WaitForAfterrunFail_s input; VPMM_TimeWaitForAfterrun_s local single; ENUM_PDUACRLYSTA_CLOSE parameter; ENUM_PDUACRLYSTA_CLOSEFAILURE parameter; ENUM_PDUACRLYSTA_OPEN parameter; ENUM_ACHVLOOP_POWEROFF parameter; ENUM_ACHVLOOP_POWERON parameter; ENUM_MCUHVLOOPSTS_PRECHARGEFIN parameter; ENUM_MCUHVLOOPSTS_OPEN parameter; ENUM_MCUHVLOOP_POWEROFF parameter; ENUM_MCUHVLOOP_POWERON parameter; VPMM_HVSelfChkCompleted4Chrg_flg local boolean; VPMM_HVSelfChkCompleted4PU_flg local boolean; VPMM_HVUnitSelfChkCompleted4PU_flg input; VPMM_TimeSysPowerOff_s local single; ENUM_MCUHVLOOPSTS_FAILED parameter; ENUM_KEYSTATUS_OFF parameter; VPMM_ExtTorquePrevent_enum output uint8; VPMM_ForcedPowerDown4IRC_flg local boolean; ENUM_PMMMODE_SLEEP parameter; KPMM_Time4Sleep_s input; KPMM_ForceEntrySleep_flg input; VPMM_PwrOffCompleted_flg local boolean size=1; VPMM_HVUnitSelfChkCompleted4Chrg_flg input; VPMM_VCUMCUCtrlMd_enum output uint8; VINP_MCUFailGrade_enum input; VPMM_VCUMCUEn_flg output boolean; KPMM_MCUEnableFailtime_s input; VPMM_MCUDisChrgFail_flg local boolean; VPMM_MCUEnableCompleted_flg local boolean; VPMM_TimeMCUEnable_s local single; ENUM_MCUCTRLMODE_ACTDISCHRG parameter; ENUM_MCUCTRLMODE_NONE parameter; ENUM_PMMMODE_INITIALIZE parameter; ENUM_TORQUEPRVENT_NOREQUEST parameter; ZERO_INT parameter; ENUM_PUFAULT_MCUENABLEFAIL parameter; VPMM_NoAfterRunRequest_flg local boolean; VPMM_AfterrunCompleted_flg local boolean; VPMM_TimeDCDCRlyDemDelay_s local single; KPMM_DCDCRlyDemDelayTime_s input; KPMM_PDULoadRlyPUFailtime_s input; VPMM_TimePDULoadRlyPU_s local single; VPMM_HVPwrFail_flg local boolean; KPMM_WaitAirPressTimeout_s input; VPMM_EHPSEACReady_flg local boolean; KPMM_AfterrunTimeout_s input; VPMM_ForceOffInAfterun_flg local boolean; VPMM_TimeForceOffInAfterrun_s local single; VPMM_HVILEmergencyStop_flg input; VTHC_AfterrunningMode_flg input; ENUM_PUFAULT_AIRPRESS parameter; ENUM_PUFAULT_EHPSENABLEFAIL parameter; ENUM_PUSTATE_DCDCRLYCLOSED parameter; ENUM_PUSTATE_PDURLYCLOSED parameter; KPMM_ButtonHoldlimit_cnt input; VINP_PushButton_flg input; VPMM_ButtonHoldtime_cnt local single; KPMM_ChrgwakeDebon_cnt input; VPMM_ChrgwakeDebon_cnt local uint8; VPMM_SSBrisdetect_flg input; VPMM_SSBrisevent_flg local boolean; VPMM_ChrgIGNTrig_flg local boolean; ENUM_PUFAULT_HVRLYCHKFAIL parameter; ENUM_PUSTATE_DRIVESAFE parameter; ENUM_PUSTATE_DCDCENABLE parameter; ENUM_PUSTATE_EHPSENABLE parameter; ENUM_PUSTATE_PDUMCURLYCLOSED parameter; ENUM_PUSTATE_MCUENABLE parameter; ENUM_PUSTATE_EACPRESCHECK parameter; VPMM_MCUPrechrgProc_flg output boolean; VPMM_MCUEnableProc_flg output boolean; VPMM_DCDCEnableProc_flg output boolean; VPMM_EHPSEnableProc_flg output boolean; VPMM_CACPresReadyProc_flg output boolean; ENUM_CACENABLESTS_FAULT parameter; ENUM_EHPSENABLESTS_FAULT parameter; VINP_PDUMCUPosRlySta_enum input; VINP_PDUACRlySta_enum input; ENUM_ACMAINRLYSTS_OPEN parameter; ENUM_MCUMAINRLYSTS_OPEN parameter; VPMM_TimeHVRlyOpen_s local single; VPMM_MCUEnDischrgCompleted_flg local boolean; KPMM_HVRlyOpenFailtime_s input; KPMM_MCUEnDischrgFailtime_s input; KPMM_TargetEnDischrgVolt_V input; KPMM_MCUPassDisChrg_s input; KPMM_TargetPassDischrgVolt_V input; VPMM_MCUEnDischrgFail_flg local boolean; VPMM_TimeMCUPassDisChrg_s local single; VPMM_TimeMCUEnDisChrg_s local single; VPMM_TimeMCUDisable_s local single; ENUM_PDFAULT_ACRLYOPEN parameter; ENUM_PDFAULT_BCUDISABLE parameter; ENUM_PDFAULT_DCDCDISABLE parameter; ENUM_PDFAULT_DCDCRLYOPEN parameter; ENUM_PDFAULT_EACDISABLE parameter; ENUM_PDFAULT_EACRLYOPEN parameter; ENUM_PDFAULT_EHPSDISABLE parameter; ENUM_PDFAULT_EHPSRLYOPEN parameter; ENUM_PDFAULT_MCUDISABLE parameter; ENUM_PDFAULT_MCURLYOPEN parameter; ENUM_PDSTATE_BCUNEGRLUFS parameter; ENUM_PDSTATE_BCUPWRDOWN parameter; ENUM_PDSTATE_FSCOMPLETED parameter; ENUM_PDSTATE_MCUDISABLE parameter; ENUM_PDSTATE_MCUDISCHRG parameter; ENUM_PDSTATE_MCUDISCHRGFS parameter; ENUM_PDSTATE_MCUPASSDISCHRG parameter; ENUM_PDSTATE_PDCOMPLETED parameter; ENUM_PDSTATE_PDUDISABLE parameter; ENUM_PDSTATE_PDURLYOPEN parameter; VPMM_TimePDUDisable_s local single; VPMM_TimePDUDisableWait_s local single; VPMM_TimeHVRlyOpenWait_s local single; VPMM_MCUPassDischrgFinish_flg local boolean; VPMM_MCUDisableCompleted_flg local boolean; VPMM_MCUEnDischrgFailCom_flg local boolean; VPMM_MCUEnDischrgFinish_flg local boolean; VPMM_MCUEnFailDis_flg local boolean; VPMM_PDUDisableCompleted_flg local boolean; VPMM_PDURLYOpenFail_flg local boolean; VPMM_PDURLYOpenFinish_flg local boolean; VPMM_HVFailureChkPass_flg input boolean; VINP_PEUSelfChkSts_enum input uint8; ENUM_BMSCHRGSTS_CHARGING parameter; ENUM_CHRGFAULT_ACRLYFAIL parameter; ENUM_CHRGFAULT_BCUHVFAIL parameter; ENUM_CHRGFAULT_PDUHVFAIL parameter; ENUM_CHRGSTATE_ACRLYCLOSED parameter; ENUM_CHRGSTATE_BCUNEGRLYCLOSED parameter; ENUM_CHRGSTATE_CHECKHVRLYOPEN parameter; ENUM_CHRGSTATE_CHKCHRGSTA parameter; ENUM_CHRGSTATE_DCDCENABLE parameter; ENUM_CHRGSTATE_DCDCRLYCLOSED parameter; ENUM_CHRGSTATE_ERROR parameter; ENUM_PEUSELFCHKSTS_NOFAULT parameter; VPMM_CheckChrgStaFail_flg local boolean; VPMM_CheckChrgSta_flg local boolean; VPMM_ChrgFinishComplete_flg local boolean; VPMM_ChrgIntoPwrdown_flg local boolean; VPMM_DCDCNotEnaInChrg_flg local boolean; ENUM_CHRGFAULT_BCUNEGFAIL parameter; ENUM_CHRGFAULT_BCUTIMEOUT parameter; ENUM_CHRGFAULT_DCDCENABLE parameter; ENUM_CHRGFAULT_DCDCRLYFAIL parameter; ENUM_CHRGFAULT_HVILFAIL parameter; ENUM_CACENABLESTS_INITIAL parameter; ENUM_CACENABLESTS_READY parameter; ENUM_DCDCENABLESTS_INITIAL parameter; ENUM_DCDCENABLESTS_READY parameter; ENUM_EHPSENABLESTS_INITIAL parameter; VPMM_SysInitialTO_flg local boolean; VPMM_EACDisableFail_flg local boolean; VPMM_DCDCRlyOpenFail_flg local boolean; VPMM_DCDCDisableFail_flg local boolean; VPMM_EACRlyOpenFail_flg local boolean; VPMM_EHPSDisableFail_flg local boolean; VPMM_EHPSRlyOpenFail_flg local boolean; VPMM_MainRlyOpenFail_flg local boolean; VPMM_PDURLYOpenFinishFM_flg local boolean; VPMM_ACRlyOpenFail_flg local boolean; VPMM_ChrgPEUFail_flg local boolean; VPMM_TimeBCUGetChrg_s local single; VPMM_TimeChrgIntoPwrdownWait_s local single; VPMM_TimeDCDCChrgNotEna_s local single; task_time_s input; KPMM_BCUGetChrgTO_s input; KPMM_ChrgIntoPwrdownWait_s input; KPMM_HVRlyOpenFailWT_s input; KPMM_MCUDisChrgFSFailtime_s input; KPMM_MCUDisableFailtime_s input; KPMM_PDUDisableFailtime_s input; KPMM_PDUDisableWaitime_s input; VPMM_PDULoadPUFault_enum local uint8; ENUM_PMMMODE_STANDBY parameter; VPSA_AlcLockPass_flg input; VPMM_TimeAlcLockCheck_s local single; VPMM_AlcLockCheckCompleted_flg local boolean; ENUM_PUFAULT_ALINTERLOCK parameter; KPMM_AlcLockCheckFailtime_s input; VPMM_PDURelayPUReady_flg local boolean; KPMM_EHPSENTimeout_s input; KPMM_EHPSIniTimeout_s input; KPMM_EHPSSpdDem_rpm input; VPMM_EHPSIniReady_flg input; VPMM_PMMEACEnableDem_flg output boolean; VPMM_PMMEHPSDemSpd_rpm output single; VPMM_PMMEHPSEnableDem_flg output boolean; VPMM_EHPSEnableCompleted_flg local boolean; VPMM_TimeEACEnable_s local single; VPMM_TimeEHPSEnable_s local single; VPMM_TimeEHPSIni_s local single; KPMM_EACENTimeout_s input; VPMM_AirPressReady_flg local boolean; VPMM_TimeWaitAirPress_s local single; VPMM_EHPSIniFinish_flg output boolean; VPMM_DCDCEnableCompleted_flg local boolean; VPMM_EACEnableCompleted_flg output boolean; VPMM_MCUSta2Lost_flg input; VPMM_AtvDisChgEnFbk_flg input; ENUM_HVPWROFFREQ_POWEROFF parameter; VPMM_ChrgPowerUpFail_flg output boolean; VPMM_ChrgBCUHVFail_flg output boolean; VPMM_Boot2Initialize_flg input boolean; VPMM_AfterRun2Initialize_flg input boolean; VPMM_Initialize2Idle_flg input boolean; VPMM_Initialize2Charge_flg input boolean; VPMM_Initialize2PowerUp_flg input boolean; VPMM_PowerUp2PowerDown_flg input boolean; VPMM_Drive2PowerDown_flg input boolean; VPMM_Charge2PowerDown_flg input boolean; VDMM_DTCMCUCtrlMdNoFB_flg input boolean; VDMM_DTCBMSRlyNoFB_flg input boolean; VPMM_LVChrgPreActFinished_flg input boolean; VPMM_LVChrgInit2PowerUp_flg input boolean; ENUM_PMMMODE_LVBATCHRG parameter; VPMM_LVChrgDCDCDis_flg input boolean; VPMM_LVChrgFinished_flg input boolean; VINP_ParkBrakeSW_flg input; VINP_VCUBattVol_v input; KPMM_VoltForceOffInAfferun_v parameter; VPMM_AtvDisChgEnFbkLatch_flg local boolean; KPSA_FakeWakeRESETRising_flg input boolean size=1
